simulink model "AEB_Gateway_Only"  (Simulink 9.2)
settings: Solver=FixedStepDiscrete  StartTime=0.0  StopTime=inf  FixedStep=0.05  RelTol=1e-3
PostLoadFcn:
  | , if any(exist('dsrtsu_mdlpostloadfcn', 'file') == [2, 3, 6]), try dsrtsu_mdlpostloadfcn('Execute', bdroot); catch fprintf('Error in PostLoadFcn (dsrtsu_mdlpostloadfcn) for model "%s":\n %s\n', bdroot, lasterr); end, end,
libraries: rtican x7
(part 1 of 2)
settings Model: DSRTSU_INTERNAL_RTI_VER=520  DSRTSU_INTERNAL_RTI_TYPE=rti1401  RTICANMMDATA=struct('GeneralSetupData',struct('modelroot','C:\Users\cordunoalbarran\Documents\dSPACE\ControlDesk\6.3\AEB_Pac_testing\AEB_shortlist','generalsettings',struct('filesettings',struct('destfolder',struct('Name','RTICANMM_FILES','Check',1),'buildfolder',struct('Name','.','Check',1),'AbsDestfolder',struct('Name','C:\Users\cordunoalbarran\Documents\dSPACE\ControlDesk\6.3\AEB_Pac_testing\AEB_shortlist\RTICANMM_FILES'),'AbsBuildfolder',struct('Name','C:\Users\cordunoalbarran\Documents\dSPACE\ControlDesk\6.3\AEB_Pac_testing\AEB_shortlist'))),'options',struct('addpaths',1,'rmpaths',1,'addtrcexclusion',logical(1),'cannavigator',struct('checkmonitoring',0),'show_usrtrc',0,'use_usrtrc',0),'advanced',struct('options',ones(1,100)),'MPSetup',{{}},'RTI',struct('Type','RTI1401','Ver','7.10','Date','02-May-2018'),'modelname','AEB_Gateway_Only','block','AEB_Gateway_Only'))  DSRTSU_INTERNAL_RTIFPGA=110  Creator=ffearon  LastModifiedBy=cordunoalbarran
settings DataIOCC: LimitDataPoints=off  SaveFormat=Dataset  SignalLoggingSaveFormat=Dataset
settings OptimizationCC: BlockReduction=off  LifeSpan=auto
settings DebuggingCC: UnderspecifiedInitializationDetection=Simplified  MergeDetectMultiDrivingBlocksExec=error  FcnCallInpInsideContextMsg=error  StateNameClashWarn=none  SFUnexpectedBacktrackingDiag=error  SFNoUnconditionalDefaultTransitionDiag=error  SFExecutionAtInitializationDiag=warning
settings HardwareCC: ProdLargestAtomicInteger=Integer  ProdLargestAtomicFloat=Float  ProdIntDivRoundTo=Zero  ProdEndianess=BigEndian  ProdHWDeviceType=Custom Processor->Custom  TargetIntDivRoundTo=Zero  TargetEndianess=BigEndian  TargetHWDeviceType=Custom Processor->Custom
settings ModelReferenceCC: PropagateSignalLabelsOutOfModel=on
settings SFSimCC: SimUseLocalCustomCode=on  MATLABDynamicMemAlloc=off
settings RTWCC: SystemTargetFile=rti1401.tlc  MakeCommand=make_rti  TemplateMakefile=rti1401.tmf  Description=dSPACE DS1401 Hardware Platform  RTWUseLocalCustomCode=on
settings CodeAppCC: StateflowObjectComments=off
settings STFCustomTargetCC: ParMdlRefBuildCompliant=on  GRTInterface=off  SystemTargetFile=rti1401.tlc
settings GRTTargetCC: CompOptLevelCompliant=off  ConcurrentExecutionCompliant=off  GeneratePreprocessorConditionals=Use local settings  MatFileLogging=off  CPPClassGenCompliant=off  GRTInterface=off  UseToolchainInfoCompliant=off
settings CustomProperty: DataType=RTWOptions_EnumType_C__Program Files_dSPACE RCPHIL 2018-A_MATLAB_RTI_RTI1401_TLC_rti1401_1InitialSimState  Value=RUN
settings EnumStrPairs: String=RUN
settings ConfigComp: CovMetricSettings=dwe  CovHtmlReporting=off  CovSaveCumulativeToWorkspaceVar=off  CovSaveSingleToWorkspaceVar=off  CovExternalEMLEnable=on

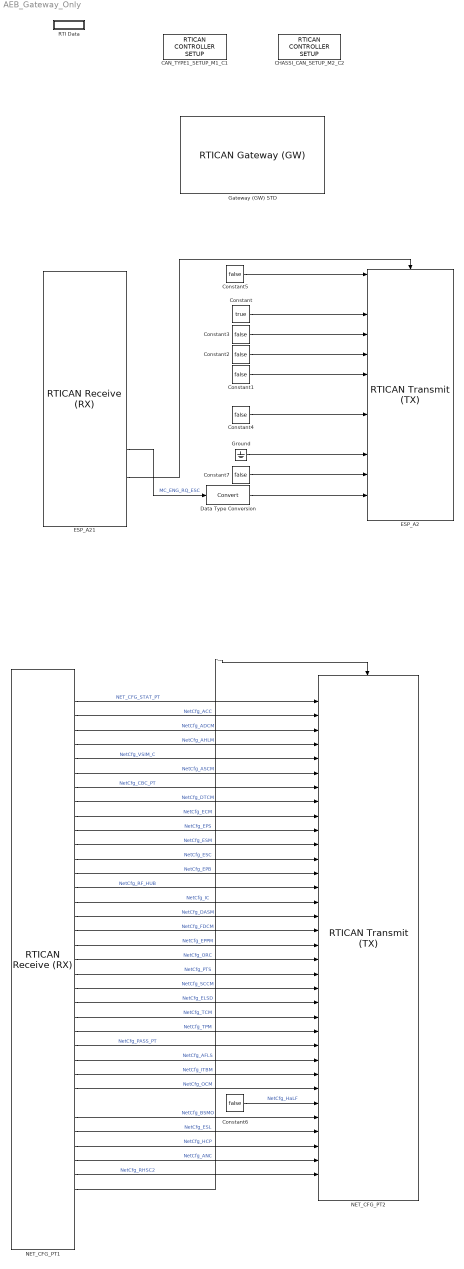
== system AEB_Gateway_Only ==
  CAN_TYPE1_SETUP_M1_C1 : rtican/RTICAN CONTROLLER SETUP   Reserved1=[]  Reserved2=[]  Reserved3=[]  Reserved4=[]  AcceptanceMask=[]  ArbitrationField=[]  Parameters=[]  SFcnRTICANSettings=[]  MS_Struct=[]  BoardTypeNo=[]  BoardNo=[]  ChannelNo=[]  DialogFcn=[]  UnitName=[]  Revision=[]  UnitValues=[]  DSProperties=struct('RTI',struct('Version',uint32(12),'BlockType',struct('isSLSource',uint8(0),'isSLSink',uint8(0),'isHWSource',uint8(0),'isHWSink',uint8(0),'isSetup',uint8(1),'isInline',uint8(1),'isNonInline',uint8(0),'isInterrupt',uint8(0),'isChannelwise',uint8(0)),'IOBoardType','RTICAN','UnitType','NON_MESSAGE','Identifier','MASTER','DialogType','ML','BlockSet','RTICAN','SlaveProcessor','CAN'))  RTIBlockInterface=struct('InputPortsWidth',int32(0),'InputPortsActive',0,'OutputPortsWidth',int32(0),'OutputPortsActive',0,'DialogFcn','rtican_master_setup_gui','BlockDisplay',{{['CAN CONTROLLER\n SETUP'],'center'}},'IconTransparency','on','InitLevel',3,'IWork',{{{'',uint32(2)}}},'BlockName',struct('Token',{{'CAN_TYPE','_SETUP_M','_C'}},'BlockParam',{{'BoardTypeNo','BoardNo','ChannelNo'}}),'ParameterTunableNames',{{}})  RTIBlockParameters="struct('BoardTypeNo',{{1,'OFF',[]}},'BoardNo',{{1,'ON',[1 16]}},'ChannelNo',{{1,'ON',[1 2]}},'AcceptanceMask',{{0,'OFF',[]}},'ArbitrationField',{{0,'OFF',[]}},'Parameters',{{struct('Config',struct('Baudrate',500,'SampleMode',1,'UsedParamSet',1,'validSettings',1,'isBTRvalues',0,'Advanced',struct('Baudrate',{500,500,500},'Frequency',{24000000,36000000,64000000},'Settings',{struct('SMPL',0,'BRP',0,'NBT',24,'TSEG1',15,'TSEG2',6,'SJW',3,'SP',70),struct('SMPL',0,'BRP',1,'NBT',18,'TSEG1',14,'TSEG2',1,'SJW',1,'SP',88),struct('SMPL',0,'BRP',3,'NBT',16,'TSEG1',12,'TSEG2',1,'SJW',1,'SP',87)},'BTR0',{192,65,67},'BTR1',{111,30,28})),'configType',1,'Options',struct('DataFileSelected',1,'DataFileName',{{['..\\..\\..\\..\\..\\..\\..\\..\\intrepidcs\\pacifica dbc\\e4a_r4_ccan_cr11690_mod.dbc']}},'DataFileDate',{{['26-Feb-2019 09:25:05']}},'InterfaceFcn','rtican_dbc_file_parser','InterfaceFcnFileName','','LabelConfigType','volatile','AcceptanceMaskSelected',0,'MsgDataType','SgnSpecification','NumType','hex','MaskType','STD','AcceptanceMask',0,'ArbitrationField',0,'UseMultipleMessageAccess',1),'RxReceiveStdOptions',struct('RxServiceStdEnabled',1,'RxServiceStdMsgIdent',1000,'RxServiceStdIdentNumType',1,'RxServiceStdIdentMask',0,'RxServiceStdMaskNumType',1,'RxServiceStdQueueSize',256),'RxReceiveXtdOptions',struct('RxServiceXtdEnabled',0,'RxServiceXtdMsgIdent',1001,'RxServiceXtdIdentNumType',1,'RxServiceXtdIdentMask',0,'RxServiceXtdMaskNumType',1,'RxServiceXtdQueueSize',64),'PartialNetworkingOptions',struct('switchedon',0,'format',1,'idmask',['    XXXXX XXXXXXXX XXXXXXXX XXXXXXXX'],'idcode','0','idfilter','0','datamaskused',0,'datalength',1,'datamask','0x0000000000000000','partialnetworkenable',0),'general',struct('Termination_common',1,'Termination_C252',1,'BusConfigurationRegister',0,'Transceiver','ISO11898','isFromLib',0)),'OFF',[]}},'CCPParameters',{{struct('CRO',struct('Format','STD','NumFormat','hex','Id',1639),'DTO',struct('Format','STD','NumFormat','hex','Id',2017),'StationAdr',struct('NumFormat','hex','Value',57),'StationId',struct('Value',['dSPACE CCP Service']),'Enabled',0),'OFF',[]}},'XCPParameters',{{struct('MASTER',struct('Format','STD','NumFormat','hex','Id',256),'SLAVE',struct('Format','STD','NumFormat','hex','Id',510),'Enabled',0,'PIDTransmissionEnabled',0),'OFF',[]}},'GroupId',{{struct('Group',{{'RTICAN'}},'No',1,'Behavior',{{'EVER'}},'BlockType',{{'SOURCE'}},'NameChangeFlag',1),'OFF',[]}},'SFcnRTICANSettings',{{struct('Baudrate',500,'configType',1,'AdvancedConfig',struct('Frequency',{},'BTR0',{},'BTR1',{}),'UsedParamSet',1,'STDMaskSelected','no','XTDMaskSelected','no','BoardType','DS1','BoardNo',1,'ControllerNo',1,'Transceiver','ISO11898','BusConfigRegister',0,'TerminationRes',120,'UseMultipleMessageAccess','yes','STDRXSrvcUsed','yes','STDRXSrvcMsgId',1,'STDRXSrvcMsgMask',0,'STDRXSrvcQueueSize',256,'XTDRXSrvcUsed','no','XTDRXSrvcMsgId',1001,'XTDRXSrvcQueueSize',64,'XTDRXSrvcMsgMask',0,'PN_IsPNTransciever',0,'PN_IsPNEnabled',0,'PN_MsgFormat',1,'PN_idcode',0,'PN_idmask',2047,'PN_datamaskused',0,'PN_datalength',0,'PN_datamask',['0xFF, 0xFF, 0xFF, 0xFF, 0xFF, 0xFF, 0xFF, 0xFF']),'OFF',[]}},'SFcnRTICCPSettings',{{struct('CRO',struct('Format','STD','NumFormat','hex','Id',1639),'DTO',struct('Format','STD','NumFormat','hex','Id',2017),'StationAdr',struct('NumFormat','hex','Value',57),'StationId',struct('Value',['dSPACE CCP Service']),'Enabled',0),'OFF',[]}},'SFcnRTIXCPSettings',{{struct('MASTER',struct('Format','STD','NumFormat','hex','Id',256),'SLAVE',struct('Format','STD','NumFormat','hex','Id',510),'Enabled',0,'PIDTransmissionEnabled',0),'OFF',[]}},'TLCFileName',{{'rtican_master_setup','OFF',[]}})"  RTISFcnParameters=struct('SFcnRTICANSettings','struct','SFcnRTICCPSettings','struct','SFcnRTIXCPSettings','struct','AcceptanceMask','int32','ArbitrationField','int32','TLCFileName','char')  RTIBlockParaDefault="struct('BoardTypeNo',4302,'BoardNo',1,'ChannelNo',1,'AcceptanceMask',0,'ArbitrationField',0,'Parameters',struct('Config',struct('Baudrate',500,'SampleMode',1,'UsedParamSet',1,'validSettings',1,'isBTRvalues',0,'Advanced',struct('Frequency',16000000,'BTR0',64,'BTR1',28,'Settings',struct('SMPL',0,'BRP',0,'NBT',16,'TSEG1',12,'TSEG2',1,'SJW',1,'SP',87))),'configType',1,'Options',struct('DataFileSelected',0,'DataFileName',{{['<no datafile support>']}},'DataFileDate',{{''}},'InterfaceFcn','rtican_dbc_file_parser','InterfaceFcnFileName','','LabelConfigType','volatile','AcceptanceMaskSelected',0,'MsgDataType','AllwaysDouble','NumType','hex','MaskType','STD','AcceptanceMask',0,'ArbitrationField',0,'UseMultipleMessageAccess',0),'RxReceiveStdOptions',struct('RxServiceStdEnabled',0,'RxServiceStdMsgIdent',1000,'RxServiceStdIdentNumType',1,'RxServiceStdIdentMask',0,'RxServiceStdMaskNumType',1,'RxServiceStdQueueSize',64),'RxReceiveXtdOptions',struct('RxServiceXtdEnabled',0,'RxServiceXtdMsgIdent',1001,'RxServiceXtdIdentNumType',1,'RxServiceXtdIdentMask',0,'RxServiceXtdMaskNumType',1,'RxServiceXtdQueueSize',64),'PartialNetworkingOptions',struct('switchedon',0,'format',1,'idmask',['    XXXXX XXXXXXXX XXXXXXXX XXXXXXXX'],'idcode','0','idfilter','0','datamaskused',0,'datalength',1,'datamask','0x0000000000000000','partialnetworkenable',0),'general',struct('Termination_common',1,'Termination_C252',1,'BusConfigurationRegister',0,'Transceiver','ISO11898','isFromLib',1)),'CCPParameters',struct('CRO',struct('Format','STD','NumFormat','hex','Id',1639),'DTO',struct('Format','STD','NumFormat','hex','Id',2017),'StationAdr',struct('NumFormat','hex','Value',57),'StationId',struct('Value',['dSPACE CCP Service']),'Enabled',0),'XCPParameters',struct('MASTER',struct('Format','STD','NumFormat','hex','Id',256),'SLAVE',struct('Format','STD','NumFormat','hex','Id',510),'Enabled',0,'PIDTransmissionEnabled',0),'GroupId',struct('Group',{{'RTICAN'}},'No',1,'Behavior',{{'EVER'}},'BlockType',{{'SOURCE'}},'NameChangeFlag',1),'SFcnRTICANSettings',struct('Baudrate',500,'configType',1,'AdvandedConfig',struct('Frequency',16000000,'BTR0','0x40','BTR1','0x1C'),'UsedParamSet',1,'STDMaskSelected','no','XTDMaskSelected','no','BoardType','DS4302','BoardNo',1,'ControllerNo',1,'Transceiver','ISO11898','BusConfigRegister',0,'TerminationRes',120,'UseMultipleMessageAccess','no','STDRXSrvcUsed','no','STDRXSrvcMsgId',1000,'STDRXSrvcMsgMask',0,'STDRXSrvcQueueSize',64,'XTDRXSrvcUsed','no','XTDRXSrvcMsgId',1001,'XTDRXSrvcQueueSize',64,'XTDRXSrvcMsgMask',0),'SFcnRTICCPSettings',struct('CRO',struct('Format','STD','NumFormat','hex','Id',1639),'DTO',struct('Format','STD','NumFormat','hex','Id',2017),'StationAdr',struct('NumFormat','hex','Value',57),'StationId',struct('Value',['dSPACE CCP Service']),'Enabled',0),'SFcnRTIXCPSettings',struct('MASTER',struct('Format','STD','NumFormat','hex','Id',256),'SLAVE',struct('Format','STD','NumFormat','hex','Id',510),'Enabled',0,'PIDTransmissionEnabled',0),'TLCFileName','rtican_master_setup')"
      settings: AttributesFormatString=Group Id: RTICAN1\n  SourceProductName=dSPACE RTI CAN Blockset
  CHASSI_CAN_SETUP_M2_C2 : rtican/RTICAN CONTROLLER SETUP   Reserved1=[]  Reserved2=[]  Reserved3=[]  Reserved4=[]  AcceptanceMask=[]  ArbitrationField=[]  Parameters=[]  SFcnRTICANSettings=[]  MS_Struct=[]  BoardTypeNo=[]  BoardNo=[]  ChannelNo=[]  DialogFcn=[]  UnitName=[]  Revision=[]  UnitValues=[]  DSProperties=struct('RTI',struct('Version',uint32(12),'BlockType',struct('isSLSource',uint8(0),'isSLSink',uint8(0),'isHWSource',uint8(0),'isHWSink',uint8(0),'isSetup',uint8(1),'isInline',uint8(1),'isNonInline',uint8(0),'isInterrupt',uint8(0),'isChannelwise',uint8(0)),'IOBoardType','RTICAN','UnitType','NON_MESSAGE','Identifier','MASTER','DialogType','ML','BlockSet','RTICAN','SlaveProcessor','CAN'))  RTIBlockInterface=struct('InputPortsWidth',int32(0),'InputPortsActive',0,'OutputPortsWidth',int32(0),'OutputPortsActive',0,'DialogFcn','rtican_master_setup_gui','BlockDisplay',{{['CAN CONTROLLER\n SETUP'],'center'}},'IconTransparency','on','InitLevel',3,'IWork',{{{'',uint32(2)}}},'BlockName',struct('Token',{{'CAN_TYPE','_SETUP_M','_C'}},'BlockParam',{{'BoardTypeNo','BoardNo','ChannelNo'}}),'ParameterTunableNames',{{}})  RTIBlockParameters="struct('BoardTypeNo',{{1,'OFF',[]}},'BoardNo',{{2,'ON',[1 16]}},'ChannelNo',{{2,'ON',[1 2]}},'AcceptanceMask',{{0,'OFF',[]}},'ArbitrationField',{{0,'OFF',[]}},'Parameters',{{struct('Config',struct('Baudrate',500,'SampleMode',1,'UsedParamSet',1,'validSettings',1,'isBTRvalues',0,'Advanced',struct('Baudrate',{500,500,500},'Frequency',{24000000,36000000,64000000},'Settings',{struct('SMPL',0,'BRP',0,'NBT',24,'TSEG1',15,'TSEG2',6,'SJW',3,'SP',70),struct('SMPL',0,'BRP',1,'NBT',18,'TSEG1',14,'TSEG2',1,'SJW',1,'SP',88),struct('SMPL',0,'BRP',3,'NBT',16,'TSEG1',12,'TSEG2',1,'SJW',1,'SP',87)},'BTR0',{192,65,67},'BTR1',{111,30,28})),'configType',1,'Options',struct('DataFileSelected',1,'DataFileName',{{['..\\..\\..\\..\\..\\..\\..\\..\\intrepidcs\\pacifica dbc\\e4a_r4_ccan_cr11690_mod.dbc']}},'DataFileDate',{{['26-Feb-2019 09:25:05']}},'InterfaceFcn','rtican_dbc_file_parser','InterfaceFcnFileName','','LabelConfigType','volatile','AcceptanceMaskSelected',0,'MsgDataType','SgnSpecification','NumType','hex','MaskType','STD','AcceptanceMask',0,'ArbitrationField',0,'UseMultipleMessageAccess',1),'RxReceiveStdOptions',struct('RxServiceStdEnabled',1,'RxServiceStdMsgIdent',1000,'RxServiceStdIdentNumType',1,'RxServiceStdIdentMask',0,'RxServiceStdMaskNumType',1,'RxServiceStdQueueSize',256),'RxReceiveXtdOptions',struct('RxServiceXtdEnabled',0,'RxServiceXtdMsgIdent',1001,'RxServiceXtdIdentNumType',1,'RxServiceXtdIdentMask',0,'RxServiceXtdMaskNumType',1,'RxServiceXtdQueueSize',64),'PartialNetworkingOptions',struct('switchedon',0,'format',1,'idmask',['    XXXXX XXXXXXXX XXXXXXXX XXXXXXXX'],'idcode','0','idfilter','0','datamaskused',0,'datalength',1,'datamask','0x0000000000000000','partialnetworkenable',0),'general',struct('Termination_common',1,'Termination_C252',1,'BusConfigurationRegister',0,'Transceiver','ISO11898','isFromLib',0)),'OFF',[]}},'CCPParameters',{{struct('CRO',struct('Format','STD','NumFormat','hex','Id',1639),'DTO',struct('Format','STD','NumFormat','hex','Id',2017),'StationAdr',struct('NumFormat','hex','Value',57),'StationId',struct('Value',['dSPACE CCP Service']),'Enabled',0),'OFF',[]}},'XCPParameters',{{struct('MASTER',struct('Format','STD','NumFormat','hex','Id',256),'SLAVE',struct('Format','STD','NumFormat','hex','Id',510),'Enabled',0,'PIDTransmissionEnabled',0),'OFF',[]}},'GroupId',{{struct('Group',{{'RTICAN'}},'No',3,'Behavior',{{'EVER'}},'BlockType',{{'SOURCE'}},'NameChangeFlag',1),'OFF',[]}},'SFcnRTICANSettings',{{struct('Baudrate',500,'configType',1,'AdvancedConfig',struct('Frequency',{},'BTR0',{},'BTR1',{}),'UsedParamSet',1,'STDMaskSelected','no','XTDMaskSelected','no','BoardType','DS1','BoardNo',2,'ControllerNo',2,'Transceiver','ISO11898','BusConfigRegister',0,'TerminationRes',120,'UseMultipleMessageAccess','yes','STDRXSrvcUsed','yes','STDRXSrvcMsgId',1,'STDRXSrvcMsgMask',0,'STDRXSrvcQueueSize',256,'XTDRXSrvcUsed','no','XTDRXSrvcMsgId',1001,'XTDRXSrvcQueueSize',64,'XTDRXSrvcMsgMask',0,'PN_IsPNTransciever',0,'PN_IsPNEnabled',0,'PN_MsgFormat',1,'PN_idcode',0,'PN_idmask',2047,'PN_datamaskused',0,'PN_datalength',0,'PN_datamask',['0xFF, 0xFF, 0xFF, 0xFF, 0xFF, 0xFF, 0xFF, 0xFF']),'OFF',[]}},'SFcnRTICCPSettings',{{struct('CRO',struct('Format','STD','NumFormat','hex','Id',1639),'DTO',struct('Format','STD','NumFormat','hex','Id',2017),'StationAdr',struct('NumFormat','hex','Value',57),'StationId',struct('Value',['dSPACE CCP Service']),'Enabled',0),'OFF',[]}},'SFcnRTIXCPSettings',{{struct('MASTER',struct('Format','STD','NumFormat','hex','Id',256),'SLAVE',struct('Format','STD','NumFormat','hex','Id',510),'Enabled',0,'PIDTransmissionEnabled',0),'OFF',[]}},'TLCFileName',{{'rtican_master_setup','OFF',[]}})"  RTISFcnParameters=struct('SFcnRTICANSettings','struct','SFcnRTICCPSettings','struct','SFcnRTIXCPSettings','struct','AcceptanceMask','int32','ArbitrationField','int32','TLCFileName','char')  RTIBlockParaDefault="struct('BoardTypeNo',4302,'BoardNo',1,'ChannelNo',1,'AcceptanceMask',0,'ArbitrationField',0,'Parameters',struct('Config',struct('Baudrate',500,'SampleMode',1,'UsedParamSet',1,'validSettings',1,'isBTRvalues',0,'Advanced',struct('Frequency',16000000,'BTR0',64,'BTR1',28,'Settings',struct('SMPL',0,'BRP',0,'NBT',16,'TSEG1',12,'TSEG2',1,'SJW',1,'SP',87))),'configType',1,'Options',struct('DataFileSelected',0,'DataFileName',{{['<no datafile support>']}},'DataFileDate',{{''}},'InterfaceFcn','rtican_dbc_file_parser','InterfaceFcnFileName','','LabelConfigType','volatile','AcceptanceMaskSelected',0,'MsgDataType','AllwaysDouble','NumType','hex','MaskType','STD','AcceptanceMask',0,'ArbitrationField',0,'UseMultipleMessageAccess',0),'RxReceiveStdOptions',struct('RxServiceStdEnabled',0,'RxServiceStdMsgIdent',1000,'RxServiceStdIdentNumType',1,'RxServiceStdIdentMask',0,'RxServiceStdMaskNumType',1,'RxServiceStdQueueSize',64),'RxReceiveXtdOptions',struct('RxServiceXtdEnabled',0,'RxServiceXtdMsgIdent',1001,'RxServiceXtdIdentNumType',1,'RxServiceXtdIdentMask',0,'RxServiceXtdMaskNumType',1,'RxServiceXtdQueueSize',64),'PartialNetworkingOptions',struct('switchedon',0,'format',1,'idmask',['    XXXXX XXXXXXXX XXXXXXXX XXXXXXXX'],'idcode','0','idfilter','0','datamaskused',0,'datalength',1,'datamask','0x0000000000000000','partialnetworkenable',0),'general',struct('Termination_common',1,'Termination_C252',1,'BusConfigurationRegister',0,'Transceiver','ISO11898','isFromLib',1)),'CCPParameters',struct('CRO',struct('Format','STD','NumFormat','hex','Id',1639),'DTO',struct('Format','STD','NumFormat','hex','Id',2017),'StationAdr',struct('NumFormat','hex','Value',57),'StationId',struct('Value',['dSPACE CCP Service']),'Enabled',0),'XCPParameters',struct('MASTER',struct('Format','STD','NumFormat','hex','Id',256),'SLAVE',struct('Format','STD','NumFormat','hex','Id',510),'Enabled',0,'PIDTransmissionEnabled',0),'GroupId',struct('Group',{{'RTICAN'}},'No',1,'Behavior',{{'EVER'}},'BlockType',{{'SOURCE'}},'NameChangeFlag',1),'SFcnRTICANSettings',struct('Baudrate',500,'configType',1,'AdvandedConfig',struct('Frequency',16000000,'BTR0','0x40','BTR1','0x1C'),'UsedParamSet',1,'STDMaskSelected','no','XTDMaskSelected','no','BoardType','DS4302','BoardNo',1,'ControllerNo',1,'Transceiver','ISO11898','BusConfigRegister',0,'TerminationRes',120,'UseMultipleMessageAccess','no','STDRXSrvcUsed','no','STDRXSrvcMsgId',1000,'STDRXSrvcMsgMask',0,'STDRXSrvcQueueSize',64,'XTDRXSrvcUsed','no','XTDRXSrvcMsgId',1001,'XTDRXSrvcQueueSize',64,'XTDRXSrvcMsgMask',0),'SFcnRTICCPSettings',struct('CRO',struct('Format','STD','NumFormat','hex','Id',1639),'DTO',struct('Format','STD','NumFormat','hex','Id',2017),'StationAdr',struct('NumFormat','hex','Value',57),'StationId',struct('Value',['dSPACE CCP Service']),'Enabled',0),'SFcnRTIXCPSettings',struct('MASTER',struct('Format','STD','NumFormat','hex','Id',256),'SLAVE',struct('Format','STD','NumFormat','hex','Id',510),'Enabled',0,'PIDTransmissionEnabled',0),'TLCFileName','rtican_master_setup')"
      settings: AttributesFormatString=Group Id: RTICAN3\n  SourceProductName=dSPACE RTI CAN Blockset
  Constant : Constant  Value=true
  Constant{1..7} (7 alike) : Constant  Value=false
  Data Type Conversion : DataTypeConversion
  ESP_A2 : rtican/RTICAN Transmit (TX)   Reserved1=[]  Reserved2=[]  Reserved3=[]  Reserved4=[]  SfcnMessage=[]  Msg_Struct=[]  BoardTypeNo=[]  BoardNo=[]  ChannelNo=[]  Parameters=[]  DialogFcn=[]  UnitName=[]  Revision=[]  UnitValues=[]  DSProperties=struct('RTI',struct('Version',uint32(5),'BlockType',struct('isSLSource',uint8(1),'isSLSink',uint8(1),'isHWSource',uint8(0),'isHWSink',uint8(0),'isSetup',uint8(0),'isInline',uint8(1),'isNonInline',uint8(0),'isInterrupt',uint8(0),'isChannelwise',uint8(0)),'IOBoardType','RTICAN','UnitType','MESSAGE','Identifier','TX','DialogType','MSVC','BlockSet','RTICAN','SlaveProcessor','CAN'))  RTIBlockInterface=struct('InputPortsWidth',int32([1 1 1 1 1 1 1 1 1 1 1 1 1]),'InputPortsActive',ones(1,13),'InputPortsName',{{'EngTrq_Rq_ESC','MaxTrqGrdAvail_ESC','DAS_Enbl_Rq','ASRActive','EngTrqMin_Rq_ESC','EngTrqMax_Rq_ESC','MaxTqAvail_ESC','PrefillActive','VehicleSpeed_SSM','DAS_RqActv','Brk_Jrk_Rsp','MC_ENG_RQ_ESC','CRC_ENG_RQ_ESC'}},'InputPortsDataType',{{'SS_BOOLEAN','SS_UINT16','SS_BOOLEAN','SS_BOOLEAN','SS_BOOLEAN','SS_BOOLEAN','SS_INT32','SS_BOOLEAN','SS_DOUBLE','SS_UINT8','SS_BOOLEAN','SS_UINT8','SS_UINT8'}},'OutputPortsWidth',int32([1 1 1 1]),'OutputPortsActive',[1 1 1 1],'OutputPortsName',{{['TX status'],['TX time'],['TX delta time'],['TX delay time']}},'DialogFcn','rtican_message_interface_gui','BlockDisplay',{{'','center'}},'IconTransparency','on','InitLevel',3,'BlockName',struct('Token',{{'ESP_A2'}}),'SampleTime',{{-1}},'TriggerPort',{{'none'}},'EnablePort',{{'yes'}})  RTIBlockParameters=struct('BoardTypeNo',{{1,'OFF',[]}},'BoardNo',{{2,'ON',[1 16]}},'ChannelNo',{{2,'ON',[1 2]}},'Parameters',{{struct('DataFileSupport',struct('DataFileSelectedMaster',1,'DataFileSelectedLocal',1,'DataFileName',['c:\users\cordunoalbarran\documents\repo\avcampari\guv0 dbcs\lyftctrlcan.dbc|'],'DataFileDate',['26-Feb-2019 09:25:05'],'SelectedFile',['..\..\..\..\..\..\..\..\intrepidcs\pacifica dbc\e4a_r4_ccan_cr11690_mod.dbc'],'InterfaceFcn','rtican_dbc_file_parser'),'Options',struct('StatusSelected',1,'TimeSelected',1,'DeltaTimeSelected',1,'DelayTimeSelected',1,'DelayTimeTXCommandSelected',0,'EncodeSetUnusedBitsToOne',0,'EnableMsgLoopback',0,'TriggerPort',struct('Selected',0,'TriggerType',0),'EnablePortSelected',1,'SignalOnPortnameSelected',1,'UserCoding',struct('Selected',1,'InterfaceFile','UserEncodingFile','FcnName','Message_CRC_Encoder','InportSelected',0,'InportWidth',1,'OutportSelected',0,'OutportWidth',1),'TerminationMsg',struct('Selected',0,'Byte0_7','0'),'InitialMsg',struct('Selected',0,'Byte0_7','0')),'Message',struct('MsgOnBlocknameSelected',1,'MsgName','ESP_A2','MsgIdFormat',0,'MsgId',268,'MsgLength',8,'NumSignals',13,'SampleTime',-1,'StartTime',struct('Selected',0,'Value',9),'AutoRepeatTime',struct('Selected',0,'Value',0.1),'Timeout',struct('Selected',0,'Value',0.1),'DelayTime',struct('Selected',0,'Value',0.1),'Signal',struct('SgnName',{'EngTrq_Rq_ESC','MaxTrqGrdAvail_ESC','DAS_Enbl_Rq','ASRActive','EngTrqMin_Rq_ESC','EngTrqMax_Rq_ESC','MaxTqAvail_ESC','PrefillActive','VehicleSpeed_SSM','DAS_RqActv','Brk_Jrk_Rsp','MC_ENG_RQ_ESC','CRC_ENG_RQ_ESC'},'SgnStartBit',{6,16,20,21,22,23,32,34,48,48,51,52,56},'SgnLength',{1,10,1,1,1,1,10,1,14,3,1,4,8},'ByteLayout',{0,2,0,0,0,0,2,0,2,0,0,0,0},'Factor',{1,64,1,1,1,1,64,1,2^-6,1,1,1,1},'Offset',{0,0,0,0,0,0,-65472,0,0,0,0,0,0},'SgnComment',{['DUMMY Signal Not Used on EVA'],'',['DUMMY Signal Not Used on EVA'],['Traction control is active'],['DUMMY Signal Not Used on EVA'],['DUMMY Signal Not Used on EVA'],'',['Brake prefill is active - True = [1]'],'',['DAS request active'],['Brake jerk response; True = [1]'],['Message counter'],['CRC-checksum byte 1 to 7 according to SAE J1850']},'SgnUnit',{'','Nm/s','','','','','Nm','','km/h','','','',''},'Min',{0,0,0,0,0,0,-65472,0,0,0,0,0,0},'Max',{0,65472,0,0,0,0,0,0,255.98,0,0,15,0},'SgnType',{0,0,0,0,0,0,0,0,0,0,0,0,0},'SLDataType',{'SS_BOOLEAN','SS_UINT16','SS_BOOLEAN','SS_BOOLEAN','SS_BOOLEAN','SS_BOOLEAN','SS_INT32','SS_BOOLEAN','SS_DOUBLE','SS_UINT8','SS_BOOLEAN','SS_UINT8','SS_UINT8'},'DataType',{0,0,0,0,0,0,0,0,0,0,0,0,0},'ModeValue',{-1,-1,-1,-1,-1,-1,-1,-1,-1,-1,-1,-1,-1}),'MsgIdNumFormat',0,'MsgComment',{{''}}),'Version',1.2,'general',struct('isFromLib',0)),'OFF',[]}},'GroupId',{{struct('Group',{{'RTICAN'}},'No',3,'Behavior',{{'NAMECHANGE'}},'BlockType',{{'SINK'}},'NameChangeFlag',0),'OFF',[]}},'SFcnRTICANMessage',{{struct('MsgType','TX','SFcnPortType','Scalar','MsgName','ESP_A2','MsgIdFormat','STD','MsgId',268,'MsgLength',8,'NumSignals',13,'SampleTime',-1,'StartTime',struct('Selected','no','Value',9),'AutoRepeatTime',struct('Selected','no','Value',0.1),'Timeout',struct('Selected','no','Value',0.1),'Signal',struct('SgnName',{'EngTrq_Rq_ESC','MaxTrqGrdAvail_ESC','DAS_Enbl_Rq','ASRActive','EngTrqMin_Rq_ESC','EngTrqMax_Rq_ESC','MaxTqAvail_ESC','PrefillActive','VehicleSpeed_SSM','DAS_RqActv','Brk_Jrk_Rsp','MC_ENG_RQ_ESC','CRC_ENG_RQ_ESC'},'SgnStartBit',{6,16,20,21,22,23,32,34,48,48,51,52,56},'SgnLength',{1,10,1,1,1,1,10,1,14,3,1,4,8},'ByteLayout',{['little endian'],['motorola back.'],['little endian'],['little endian'],['little endian'],['little endian'],['motorola back.'],['little endian'],['motorola back.'],['little endian'],['little endian'],['little endian'],['little endian']},'Factor',{1,64,1,1,1,1,64,1,2^-6,1,1,1,1},'Offset',{0,0,0,0,0,0,-65472,0,0,0,0,0,0},'SgnType',{'standard','standard','standard','standard','standard','standard','standard','standard','standard','standard','standard','standard','standard'},'SLDataType',{'SS_BOOLEAN','SS_UINT16','SS_BOOLEAN','SS_BOOLEAN','SS_BOOLEAN','SS_BOOLEAN','SS_INT32','SS_BOOLEAN','SS_DOUBLE','SS_UINT8','SS_BOOLEAN','SS_UINT8','SS_UINT8'},'DataType',{['unsigned int'],['unsigned int'],['unsigned int'],['unsigned int'],['unsigned int'],['unsigned int'],['unsigned int'],['unsigned int'],['unsigned int'],['unsigned int'],['unsigned int'],['unsigned int'],['unsigned int']},'ModeValue',{-1,-1,-1,-1,-1,-1,-1,-1,-1,-1,-1,-1,-1}),'StatusSelected','yes','TimeSelected','yes','DeltaTimeSelected','yes','DelayTimeSelected','yes','DelayTimeTXCommandSelected','no','EncodeSetUnusedBitsToOne','no','EnableMsgLoopback','no','TriggerPort',struct('Selected','no','TriggerType',0),'EnablePortSelected','yes','UserCoding',struct('Selected','yes','InterfaceFile','UserEncodingFile','FcnName','Message_CRC_Encoder','InportSelected','no','InportWidth',1,'OutportSelected','no','OutportWidth',1),'TerminationMsg',struct('Selected','no','Byte0','0x00','Byte1','0x00','Byte2','0x00','Byte3','0x00','Byte4','0x00','Byte5','0x00','Byte6','0x00','Byte7','0x00'),'InitialMsg',struct('Selected','no','Byte0','0x00','Byte1','0x00','Byte2','0x00','Byte3','0x00','Byte4','0x00','Byte5','0x00','Byte6','0x00','Byte7','0x00'),'BoardType','DS1','BoardNo',2,'ControllerNo',2),'OFF',[]}},'TLCFileName',{{'rtican_tx_message','OFF',[]}})  RTISFcnParameters=struct('SFcnRTICANMessage','struct','TLCFileName','char')  RTIBlockParaDefault=struct('BoardTypeNo',4302,'BoardNo',1,'ChannelNo',1,'Parameters',struct('DataFileSupport',struct('DataFileSelectedMaster',0,'DataFileSelectedLocal',0,'DataFileName','','DataFileDate','','SelectedFile',['<no file selected>']),'Options',struct('StatusSelected',1,'TimeSelected',1,'DeltaTimeSelected',1,'DelayTimeSelected',1,'DelayTimeTXCommandSelected',0,'EncodeSetUnusedBitsToOne',0,'EnableMsgLoopback',0,'TriggerPort',struct('Selected',0,'TriggerType','rising'),'EnablePortSelected',0,'SignalOnPortnameSelected',1,'UserCoding',struct('Selected',0,'InterfaceFile','UserEncodingFile','FcnName','UserEncodeFcn','InportSelected',0,'InportWidth',1,'OutportSelected',0,'OutportWidth',1),'TerminationMsg',struct('Selected',0,'Byte0_7','0'),'InitialMsg',struct('Selected',0,'Byte0_7','0')),'Message',struct('MsgOnBlocknameSelected',0,'MsgName',['TX Message'],'MsgIdFormat',0,'MsgId',100,'MsgLength',8,'NumSignals',1,'SampleTime',-1,'StartTime',struct('Selected',0,'Value',0),'AutoRepeatTime',struct('Selected',0,'Value',0.1),'Timeout',struct('Selected',0,'Value',0.1),'DelayTime',struct('Selected',0,'Value',0.1),'Signal',struct('SgnName',['TX signal'],'SgnStartBit',0,'SgnLength',8,'SgnType',0,'ModeValue',-1,'DataType',0,'SLDataType','SS_DOUBLE','ByteLayout',0,'Factor',1,'Offset',0,'Min',0,'Max',255,'SgnComment',{{}},'SgnUnit',''),'MsgIdNumFormat',0,'MsgComment',{{''}}),'Version',1.2,'general',struct('isFromLib',1)),'GroupId',struct('Group',{{'RTICAN'}},'No',1,'Behavior',{{'NAMECHANGE'}},'BlockType',{{'SINK'}},'NameChangeFlag',0),'SFcnRTICANMessage',struct('MsgType','TX','MsgName',['TX Message'],'MsgIdFormat','STD','MsgId',100,'MsgLength',2,'NumSignals',1,'SampleTime',-1,'StartTime',struct('Selected','no','Value',0),'AutoRepeatTime',struct('Selected','no','Value',0.1),'Timeout',struct('Selected','no','Value',0.1),'DelayTime',struct('Selected','no','Value',0.1),'Signal',struct('SgnName',['TX signal'],'SgnStartBit',0,'SgnLength',8,'SgnType','standard','ModeValue',-1,'DataType',['unsigned int'],'ByteLayout',['little endian'],'SLDataType','SS_DOUBLE','Factor',1,'Offset',0),'StatusSelected','yes','TimeSelected','yes','DeltaTimeSelected','yes','DelayTimeSelected','yes','EnablePortSelected','no','EnableMsgLoopback','no','DelayTimeTXCommandSelected','no','EncodeSetUnusedBitsToOne','no','UserCoding',struct('Selected','no','InterfaceFile','UserDecodingFile','FcnName','UserDecodeFcn','InportSelected','no','InportWidth',1,'OutportSelected','no','OutportWidth',1),'TerminationMsg',struct('Selected','no','Byte0','0x00','Byte1','0x00','Byte2','0x00','Byte3','0x00','Byte4','0x00','Byte5','0x00','Byte6','0x00','Byte7','0x00'),'InitialMsg',struct('Selected','no','Byte0','0x00','Byte1','0x00','Byte2','0x00','Byte3','0x00','Byte4','0x00','Byte5','0x00','Byte6','0x00','Byte7','0x00'),'TriggerPort',struct('Selected','no','TriggerType','rising'),'BoardType','DS4302','BoardNo',1,'ControllerNo',1,'SFcnPortType','Scalar'),'TLCFileName','rtican_tx_message')
      settings: AttributesFormatString=Group Id: RTICAN3\n  SourceProductName=dSPACE RTI CAN Blockset
  ESP_A21 : rtican/RTICAN Receive (RX)   Reserved1=[]  Reserved2=[]  Reserved3=[]  Reserved4=[]  SfcnMessage=[]  Msg_Struct=[]  BoardTypeNo=[]  BoardNo=[]  ChannelNo=[]  Parameters=[]  DialogFcn=[]  UnitName=[]  Revision=[]  UnitValues=[]  DSProperties=struct('RTI',struct('Version',uint32(5),'BlockType',struct('isSLSource',uint8(1),'isSLSink',uint8(1),'isHWSource',uint8(0),'isHWSink',uint8(0),'isSetup',uint8(0),'isInline',uint8(1),'isNonInline',uint8(0),'isInterrupt',uint8(0),'isChannelwise',uint8(0)),'IOBoardType','RTICAN','UnitType','MESSAGE','Identifier','RX','DialogType','MSVC','BlockSet','RTICAN','SlaveProcessor','CAN'))  RTIBlockInterface=struct('OutputPortsWidth',int32([1 1 1 1 1 1 1 1 1 1 1 1 1 1 1 1]),'OutputPortsActive',ones(1,16),'OutputPortsName',{{'EngTrq_Rq_ESC','MaxTrqGrdAvail_ESC','DAS_Enbl_Rq','ASRActive','EngTrqMin_Rq_ESC','EngTrqMax_Rq_ESC','MaxTqAvail_ESC','PrefillActive','VehicleSpeed_SSM','DAS_RqActv','Brk_Jrk_Rsp','MC_ENG_RQ_ESC','CRC_ENG_RQ_ESC',['RX status'],['RX time'],['RX delta time']}},'OutputPortsDataType',{{'SS_BOOLEAN','SS_UINT16','SS_BOOLEAN','SS_BOOLEAN','SS_BOOLEAN','SS_BOOLEAN','SS_INT32','SS_BOOLEAN','SS_DOUBLE','SS_UINT8','SS_BOOLEAN','SS_UINT8','SS_UINT8','SS_DOUBLE','SS_DOUBLE','SS_DOUBLE'}},'OutputPortsLabel',{{'EngTrq_Rq_ESC','MaxTrqGrdAvail_ESC','DAS_Enbl_Rq','ASRActive','EngTrqMin_Rq_ESC','EngTrqMax_Rq_ESC','MaxTqAvail_ESC','PrefillActive','VehicleSpeed_SSM','DAS_RqActv','Brk_Jrk_Rsp','MC_ENG_RQ_ESC','CRC_ENG_RQ_ESC','','',''}},'OutputPortsLabelMode','ON','InputPortsWidth',int32(0),'InputPortsActive',0,'DialogFcn','rtican_message_interface_gui','BlockDisplay',{{'','center'}},'IconTransparency','on','ParameterTunableNames',{{}},'InitLevel',3,'BlockName',struct('Token',{{'ESP_A2'}}),'SampleTime',{{-1}},'TriggerPort',{{'none'}},'EnablePort',{{'none'}})  RTIBlockParameters=struct('BoardTypeNo',{{1,'OFF',[]}},'BoardNo',{{1,'ON',[1 16]}},'ChannelNo',{{1,'ON',[1 2]}},'Parameters',{{struct('DataFileSupport',struct('DataFileSelectedMaster',1,'DataFileSelectedLocal',1,'DataFileName',['c:\intrepidcs\pacifica dbc\e4a_r4_ccan_cr11690_mod.dbc|'],'DataFileDate',['26-Feb-2019 09:25:05'],'SelectedFile',['..\..\..\..\..\..\..\..\intrepidcs\pacifica dbc\e4a_r4_ccan_cr11690_mod.dbc'],'InterfaceFcn','rtican_dbc_file_parser'),'Options',struct('StatusSelected',1,'TimeSelected',1,'DeltaTimeSelected',1,'BytePortSelected',0,'MessageLengthSelected',0,'TriggerPort',struct('Selected',0,'TriggerType',0),'UserCoding',struct('Selected',0,'InterfaceFile','UserDecodingFile','FcnName','UserDecodeFcn','InportSelected',0,'InportWidth',1,'OutportSelected',0,'OutportWidth',1),'EnablePortSelected',0,'SignalOnPortnameSelected',1,'UseRXService',0),'Message',struct('MsgOnBlocknameSelected',1,'MsgName','ESP_A2','MsgIdFormat',0,'MsgId',268,'MsgLength',8,'NumSignals',13,'SampleTime',-1,'Signal',struct('SgnName',{'EngTrq_Rq_ESC','MaxTrqGrdAvail_ESC','DAS_Enbl_Rq','ASRActive','EngTrqMin_Rq_ESC','EngTrqMax_Rq_ESC','MaxTqAvail_ESC','PrefillActive','VehicleSpeed_SSM','DAS_RqActv','Brk_Jrk_Rsp','MC_ENG_RQ_ESC','CRC_ENG_RQ_ESC'},'SgnStartBit',{6,16,20,21,22,23,32,34,48,48,51,52,56},'SgnLength',{1,10,1,1,1,1,10,1,14,3,1,4,8},'SgnType',{0,0,0,0,0,0,0,0,0,0,0,0,0},'ModeValue',{-1,-1,-1,-1,-1,-1,-1,-1,-1,-1,-1,-1,-1},'DataType',{0,0,0,0,0,0,0,0,0,0,0,0,0},'ByteLayout',{0,2,0,0,0,0,2,0,2,0,0,0,0},'Factor',{1,64,1,1,1,1,64,1,2^-6,1,1,1,1},'Offset',{0,0,0,0,0,0,-65472,0,0,0,0,0,0},'SgnComment',{{['DUMMY Signal Not Used on EVA']},{''},{['DUMMY Signal Not Used on EVA']},{['Traction control is active']},{['DUMMY Signal Not Used on EVA']},{['DUMMY Signal Not Used on EVA']},{''},{['Brake prefill is active - True = [1]']},{''},{['DAS request active']},{['Brake jerk response; True = [1]']},{['Message counter']},{['CRC-checksum byte 1 to 7 according to SAE J1850']}},'SgnUnit',{'','Nm/s','','','','','Nm','','km/h','','','',''},'Min',{0,0,0,0,0,0,-65472,0,0,0,0,0,0},'Max',{0,65472,0,0,0,0,0,0,255.98,0,0,15,0},'SLDataType',{'SS_BOOLEAN','SS_UINT16','SS_BOOLEAN','SS_BOOLEAN','SS_BOOLEAN','SS_BOOLEAN','SS_INT32','SS_BOOLEAN','SS_DOUBLE','SS_UINT8','SS_BOOLEAN','SS_UINT8','SS_UINT8'}),'MsgIdNumFormat',0,'MsgComment',{{''}}),'Version',1.2,'general',struct('isFromLib',0)),'OFF',[]}},'GroupId',{{struct('Group',{{'RTICAN'}},'No',1,'Behavior',{{'NAMECHANGE'}},'BlockType',{{'SINK'}},'NameChangeFlag',0),'OFF',[]}},'SFcnRTICANMessage',{{struct('MsgType','RX','SFcnPortType','Scalar','MsgName','ESP_A2','MsgIdFormat','STD','MsgId',268,'MsgLength',8,'NumSignals',13,'SampleTime',-1,'Signal',struct('SgnName',{'EngTrq_Rq_ESC','MaxTrqGrdAvail_ESC','DAS_Enbl_Rq','ASRActive','EngTrqMin_Rq_ESC','EngTrqMax_Rq_ESC','MaxTqAvail_ESC','PrefillActive','VehicleSpeed_SSM','DAS_RqActv','Brk_Jrk_Rsp','MC_ENG_RQ_ESC','CRC_ENG_RQ_ESC'},'SgnStartBit',{6,16,20,21,22,23,32,34,48,48,51,52,56},'SgnLength',{1,10,1,1,1,1,10,1,14,3,1,4,8},'SgnType',{'standard','standard','standard','standard','standard','standard','standard','standard','standard','standard','standard','standard','standard'},'ModeValue',{-1,-1,-1,-1,-1,-1,-1,-1,-1,-1,-1,-1,-1},'DataType',{['unsigned int'],['unsigned int'],['unsigned int'],['unsigned int'],['unsigned int'],['unsigned int'],['unsigned int'],['unsigned int'],['unsigned int'],['unsigned int'],['unsigned int'],['unsigned int'],['unsigned int']},'ByteLayout',{['little endian'],['motorola back.'],['little endian'],['little endian'],['little endian'],['little endian'],['motorola back.'],['little endian'],['motorola back.'],['little endian'],['little endian'],['little endian'],['little endian']},'Factor',{1,64,1,1,1,1,64,1,2^-6,1,1,1,1},'Offset',{0,0,0,0,0,0,-65472,0,0,0,0,0,0},'SLDataType',{'SS_BOOLEAN','SS_UINT16','SS_BOOLEAN','SS_BOOLEAN','SS_BOOLEAN','SS_BOOLEAN','SS_INT32','SS_BOOLEAN','SS_DOUBLE','SS_UINT8','SS_BOOLEAN','SS_UINT8','SS_UINT8'}),'StatusSelected','yes','TimeSelected','yes','DeltaTimeSelected','yes','BytePortSelected','no','MessageLengthSelected','no','TriggerPort',struct('Selected','no','TriggerType',0),'UserCoding',struct('Selected','no','InterfaceFile','UserDecodingFile','FcnName','UserDecodeFcn','InportSelected','no','InportWidth',1,'OutportSelected','no','OutportWidth',1),'EnablePortSelected','no','UseRXService','no','BoardType','DS1','BoardNo',1,'ControllerNo',1),'OFF',[]}},'TLCFileName',{{'rtican_rx_message','OFF',[]}})  RTISFcnParameters=struct('SFcnRTICANMessage','struct','TLCFileName','char')  RTIBlockParaDefault=struct('BoardTypeNo',4302,'BoardNo',1,'ChannelNo',1,'Parameters',struct('DataFileSupport',struct('DataFileSelectedMaster',0,'DataFileSelectedLocal',0,'DataFileName','','DataFileDate','','SelectedFile',['<no file selected>']),'Options',struct('StatusSelected',1,'TimeSelected',1,'DeltaTimeSelected',1,'BytePortSelected',0,'MessageLengthSelected',0,'TriggerPort',struct('Selected',0,'TriggerType','rising'),'UserCoding',struct('Selected',0,'InterfaceFile','UserDecodingFile','FcnName','UserDecodeFcn','InportSelected',0,'InportWidth',1,'OutportSelected',0,'OutportWidth',1),'EnablePortSelected',0,'SignalOnPortnameSelected',1,'UseRXService',0),'Message',struct('MsgOnBlocknameSelected',0,'MsgName',['RX Message'],'MsgIdFormat',0,'MsgId',100,'MsgLength',8,'NumSignals',1,'SampleTime',-1,'Signal',struct('SgnName',['RX signal'],'SgnStartBit',0,'SgnLength',8,'SgnType',0,'ModeValue',-1,'DataType',0,'SLDataType','SS_DOUBLE','ByteLayout',0,'Factor',1,'Offset',0,'Min',0,'Max',255,'SgnComment',{{}},'SgnUnit',''),'MsgIdNumFormat',0,'MsgComment',{{''}}),'Version',1.2,'general',struct('isFromLib',1)),'GroupId',struct('Group',{{'RTICAN'}},'No',1,'Behavior',{{'NAMECHANGE'}},'BlockType',{{'SINK'}},'NameChangeFlag',0),'SFcnRTICANMessage',struct('MsgType','RX','MsgName',['RX Message'],'MsgIdFormat','STD','MsgId',100,'MsgLength',8,'NumSignals',1,'SampleTime',-1,'Signal',struct('SgnName',['RX signal'],'SgnStartBit',0,'SgnLength',8,'SgnType','standard','ModeValue',-1,'DataType',['unsigned int'],'ByteLayout',['little endian'],'SLDataType','SS_DOUBLE','Factor',1,'Offset',0),'StatusSelected','yes','TimeSelected','yes','DeltaTimeSelected','yes','BytePortSelected','no','MessageLengthSelected','no','EnablePortSelected','no','UserCoding',struct('Selected','no','InterfaceFile','UserDecodingFile','FcnName','UserDecodeFcn','InportSelected','no','InportWidth',1,'OutportSelected','no','OutportWidth',1),'TriggerPort',struct('Selected','no','TriggerType','rising'),'UseRXService','no','BoardType','DS4302','BoardNo',1,'ControllerNo',1,'SFcnPortType','Scalar'),'TLCFileName','rtican_rx_message')
      settings: AttributesFormatString=Group Id: RTICAN1\n  SourceProductName=dSPACE RTI CAN Blockset
  Gateway (GW) STD : rtican/RTICAN Gateway (GW)  Reserved1=[]  Reserved2=[]  Reserved3=[]  Reserved4=[]  BoardTypeNo=[]  BoardNo=[]  ChannelNo=[]  BoardTypeNo2=[]  BoardNo2=[]  ChannelNo2=[]  Parameters=[]  DialogFcn=[]  UnitName=[]  Revision=[]  UnitValues=[]  DSProperties=struct('RTI',struct('Version',uint32(1),'BlockType',struct('isSLSource',uint8(1),'isSLSink',uint8(1),'isHWSource',uint8(0),'isHWSink',uint8(0),'isSetup',uint8(0),'isInline',uint8(1),'isNonInline',uint8(0),'isInterrupt',uint8(0),'isChannelwise',uint8(0)),'IOBoardType','RTICAN','UnitType','MESSAGE','Identifier','GW','DialogType','MSVC','BlockSet','RTICAN','SlaveProcessor','CAN'))  RTIBlockInterface=struct('OutputPortsWidth',int32([1 1 1 1]),'OutputPortsActive',[1 1 1 1],'OutputPortsName',{{['RX count 1'],['TX count 1'],['RX count 2'],['TX count 2']}},'OutputPortsDataType',{{'SS_DOUBLE','SS_DOUBLE','SS_DOUBLE','SS_DOUBLE'}},'OutputPortsLabel',{{'','','',''}},'OutputPortsLabelMode','off','InitLevel',3,'DialogFcn','rtican_gateway_interface_gui','BlockDisplay',{{['DS1 B1 C1\n <==>\nDS1 B2 C2'],'center'}},'IconTransparency','on','IWork',{{{'',uint32(4)}}},'BlockName',struct('Token',{{['Gateway (GW) STD']}}),'SampleTime',{{-1}},'TriggerPort',{{'none'}},'EnablePort',{{'none'}})  RTIBlockParameters=struct('BoardTypeNo',{{1,'OFF',[]}},'BoardNo',{{1,'ON',[1 16]}},'ChannelNo',{{1,'ON',[1 2]}},'BoardTypeNo2',{{1,'OFF',[]}},'BoardNo2',{{2,'ON',[1 16]}},'ChannelNo2',{{2,'ON',[1 4]}},'MessageIDFormat',{{'STD','OFF',[]}},'Parameters',{{struct('SampleTime',-1,'DataFileSupport',struct('DataFileSelectedMaster',1,'DataFileSelectedLocal',0,'DataFileName',['c:\intrepidcs\pacifica dbc\e4a_r4_ccan_cr11690_mod.dbc|'],'DataFileDate','','SelectedFile',['..\..\..\..\..\..\..\..\intrepidcs\pacifica dbc\e4a_r4_ccan_cr11690_mod.dbc']),'Options',struct('RXCnt1Selected',1,'TXCnt1Selected',1,'RXCnt2Selected',1,'TXCnt2Selected',1,'BothDirSelected',1,'DiffListsSelected',1,'MsgIdFormat',0,'TriggerPort',struct('Selected',0,'TriggerType',0),'EnablePortSelected',0),'ExcludeList12',struct('Count',257,'MsgList',struct('MsgId',{969,1788,1729,1787,1784,1754,1736,1737,1786,1730,1758,1732,1762,1728,1763,838,523,524,525,998,999,927,937,520,564,861,624,456,856,848,500,499,501,625,2015,860,1900,1898,2023,2020,1568,1899,2019,2016,1882,1864,1865,2018,1858,1902,1886,1860,1890,1856,1891,1150,1260,1258,2031,2028,1284,1235,1259,2027,2024,1242,1224,1225,2026,1252,1218,1262,1246,1220,1250,1216,1251,1151,653,864,850,880,896,912,928,936,632,779,703,863,308,290,672,257,1468,1409,1427,1467,1464,1434,1416,1417,1466,1444,1410,1438,1412,1442,1408,1443,522,463,268,736,737,682,1016,989,988,987,986,985,707,714,715,1017,1018,1019,1020,1021,1022,1023,991,1008,983,982,981,980,979,706,709,710,1009,1010,1011,1012,1014,1015,984,908,974,901,639,853,854,799,798,817,579,705,678,658,729,704,654,878,560,832,782,938,939,940,941,942,943,958,959,517,515,516,518,956,926,1025,1083,1050,1031,1032,1082,1026,1024,1033,1059,464,466,469,294,542,764,766,859,532,584,900,826,608,825,671,388,448,924,656,521,929,746,857,858,1596,1537,1555,1595,1592,1562,1544,1545,1594,1572,1538,1566,1540,1570,1536,1571,879,719,557,808,773,526,527,376,698,1100,906,1004,1005,1006,1007,1099,1101,898,907,947,949,948,950,2047},'MsgName',{'AMB_TEMP_DISP','APPL_ECU_BSMO','APPL_ECU_CBC','APPL_ECU_EBCM','APPL_ECU_ECM','APPL_ECU_EPS','APPL_ECU_ESL','APPL_ECU_ESM','APPL_ECU_HCP','APPL_ECU_IC','APPL_ECU_OCM','APPL_ECU_ORC','APPL_ECU_PTS','APPL_ECU_RF_HUB','APPL_ECU_SCCM','AS_CHIME_STAT','BCM_CODE_ESL_REQUEST','BCM_CODE_TRM_REQUEST','BCM_MINICRYPT_ACK','BU_NET_CFG_INT','BU_NET_CFG_PT','BU_NET_CFG_ePT','CBC_CFG1','CBC_PT6','CBC_PT7','CBC_PT7_IBS2','CBC_PT8','CBC_VTA','COMPASS_A1','Clock_Date','DAS_A3','DAS_A3_A','DAS_A4','DAS_A5','DG_RQ_GLOBAL','DIRECT_INFO','D_RQ_AHCP','D_RQ_APM','D_RQ_BPCM','D_RQ_BSMO','D_RQ_CBC','D_RQ_EAC','D_RQ_EBCM','D_RQ_ECM','D_RQ_EPS','D_RQ_ESL','D_RQ_ESM','D_RQ_HCP','D_RQ_IC','D_RQ_OBCM','D_RQ_OCM','D_RQ_ORC','D_RQ_PTS','D_RQ_RF_HUB','D_RQ_SCCM','D_RQ_SGW','D_RS_AHCP','D_RS_APM','D_RS_BPCM','D_RS_BSMO','D_RS_CBC','D_RS_DASM','D_RS_EAC','D_RS_EBCM','D_RS_ECM','D_RS_EPS','D_RS_ESL','D_RS_ESM','D_RS_HCP','D_RS_HaLF','D_RS_IC','D_RS_OBCM','D_RS_OCM','D_RS_ORC','D_RS_PTS','D_RS_RF_HUB','D_RS_SCCM','D_RS_SGW','EBCM_C1','ECM_APPL1','ECM_APPL2','ECM_APPL3','ECM_APPL4','ECM_APPL5','ECM_APPL6','ECM_APPL7','ECM_B2','ECM_B5','ECM_B7','ECM_B8','ECM_CRUISE_MAP','ECM_GEAR','ECM_INDICATORS','ECM_SKIM_OBD','ECU_APPL_BSMO','ECU_APPL_CBC','ECU_APPL_DASM','ECU_APPL_EBCM','ECU_APPL_ECM','ECU_APPL_EPS','ECU_APPL_ESL','ECU_APPL_ESM','ECU_APPL_HCP','ECU_APPL_HaLF','ECU_APPL_IC','ECU_APPL_OCM','ECU_APPL_ORC','ECU_APPL_PTS','ECU_APPL_RF_HUB','ECU_APPL_SCCM','EPS_SDS_Resp','ESL_CODE_RESPONSE','ESP_A2','ESP_B1','ESP_B2','ESP_B5','EcuBuCfg1','EcuBuCfg10','EcuBuCfg11','EcuBuCfg12','EcuBuCfg13','EcuBuCfg14','EcuBuCfg15','EcuBuCfg16','EcuBuCfg17','EcuBuCfg2','EcuBuCfg3','EcuBuCfg4','EcuBuCfg5','EcuBuCfg6','EcuBuCfg7','EcuBuCfg8','EcuBuCfg9','EcuCfg1','EcuCfg10','EcuCfg11','EcuCfg12','EcuCfg13','EcuCfg14','EcuCfg15','EcuCfg16','EcuCfg17','EcuCfg2','EcuCfg3','EcuCfg4','EcuCfg5','EcuCfg7','EcuCfg8','EcuCfg9','GPS_POS3','GW_Dev','GW_IBS2_DATA','GW_IBS_DATA','GW_LIN_I_C1','GW_LIN_I_C1_IBS2','GW_LIN_I_C2','GW_LIN_I_C2_IBS2','GW_LIN_I_C3','GW_LIN_I_C4','GW_LIN_I_C5','HALF_HMI_STATUS','HALF_MTO_SteerControl','HALF_SWVM_CTRL','HCP_2','HCP_C1','HCP_DISP','HVAC_A2','IC_500Cyc','IC_A5','IC_TripData_1','IC_TripData_2','IC_TripData_3','IC_TripData_4','IC_TripData_5','IC_TripData_6','IC_TripData_7','IC_TripData_8','IMMO_CODE_REQUEST','IMMO_CODE_REQUEST_HCP','IMMO_CODE_RESPONSE','IMMO_CODE_RESPONSE_HCP','NAV_DATA','NET_CFG_EPT','NM_CBC','NM_EBCM','NM_EPS','NM_ESC','NM_ESL','NM_HCP','NM_IC','NM_RF_HUB','NM_SBWM','NM_SCCM','ORC_A1','ORC_A2','ORC_A4','ORC_YRS_DATA','ORC_YRS_INFO','PCM_EDR','PCM_EDR2','PN14_IBS2_DATA','PN14_IBS_DATA','PN14_STAT','PN14_STAT_IBS2','PTS_1','PTS_2','PTS_CHIME_STAT','PTS_StrCtrl','RFHUB_A1','RFHUB_A2','RFHUB_A3','RF_CHAR','RHSC_SDS_SteerControl','Radio_A3','SBW_ROT1','SDS_CBC_CMD','SDS_CBC_STAT','SD_RS_BSMO','SD_RS_CBC','SD_RS_DASM','SD_RS_EBCM','SD_RS_ECM','SD_RS_EPS','SD_RS_ESL','SD_RS_ESM','SD_RS_HCP','SD_RS_HaLF','SD_RS_IC','SD_RS_OCM','SD_RS_ORC','SD_RS_PTS','SD_RS_RF_HUB','SD_RS_SCCM','STATUS_C_ESL','STATUS_C_PTS','SWS_8','TGW_DATA_IC','TPM_A2','TRM_CODE_RESPONSE','TRM_MKP_KEY','TRNS_STAT2','Uconnect_1','VehCfg6','VehCfg8','VehCfgBu1','VehCfgBu2','VehCfgBu3','VehCfgBu4','VehCfgBu5','VehCfgBu6','VehCfgBu7','VehCfgBu8','VehCfgCSM1','VehCfgCSM1_BU','VehCfgCSM2','VehCfgCSM2_BU','WAKE_SGW'},'FromDBC',{1,1,1,1,1,1,1,1,1,1,1,1,1,1,1,1,1,1,1,1,1,1,1,1,1,1,1,1,1,1,1,1,1,1,1,1,1,1,1,1,1,1,1,1,1,1,1,1,1,1,1,1,1,1,1,1,1,1,1,1,1,1,1,1,1,1,1,1,1,1,1,1,1,1,1,1,1,1,1,1,1,1,1,1,1,1,1,1,1,1,1,1,1,1,1,1,1,1,1,1,1,1,1,1,1,1,1,1,1,1,1,1,1,1,1,1,1,1,1,1,1,1,1,1,1,1,1,1,1,1,1,1,1,1,1,1,1,1,1,1,1,1,1,1,1,1,1,1,1,1,1,1,1,1,1,1,1,1,1,1,1,1,1,1,1,1,1,1,1,1,1,1,1,1,1,1,1,1,1,1,1,1,1,1,1,1,1,1,1,1,1,1,1,1,1,1,1,1,1,1,1,1,1,1,1,1,1,1,1,1,1,1,1,1,1,1,1,1,1,1,1,1,1,1,1,1,1,1,1,1,1,1,1,1,1,1,1,1,1,1,1,1,1,1,1,1,1,1,1,1,1,1,1,1,1,1,1})),'ExcludeList21',struct('Count',0,'MsgList',struct('MsgId',0,'MsgName','empty','FromDBC',0)),'Version',1,'general',struct('isFromLib',0,'BoardType2',1,'BoardNo2',2,'ControllerNo2',2,'GroupId2',struct('Group','RTICAN','No',3))),'OFF',[]}},'GroupId',{{struct('Group',{{'RTICAN'}},'No',1,'Behavior',{{'NAMECHANGE'}},'BlockType',{{'SINK'}},'NameChangeFlag',0),'OFF',[]}},'GroupId2',{{struct('Group',{{'RTICAN'}},'No',3,'Behavior',{{'NAMECHANGE'}},'BlockType',{{'SINK'}},'NameChangeFlag',0),'OFF',[]}},'SFcnRTICANMessage',{{struct('MsgIdFormat','STD','SampleTime',-1,'RXCnt1Selected','yes','TXCnt1Selected','yes','RXCnt2Selected','yes','TXCnt2Selected','yes','BothDirSelected','yes','DiffListsSelected','yes','EnablePortSelected','no','TriggerPort',struct('Selected','no','TriggerType','rising'),'ExcludeList12',struct('Count',257,'MsgList',struct('MsgId',{969,1788,1729,1787,1784,1754,1736,1737,1786,1730,1758,1732,1762,1728,1763,838,523,524,525,998,999,927,937,520,564,861,624,456,856,848,500,499,501,625,2015,860,1900,1898,2023,2020,1568,1899,2019,2016,1882,1864,1865,2018,1858,1902,1886,1860,1890,1856,1891,1150,1260,1258,2031,2028,1284,1235,1259,2027,2024,1242,1224,1225,2026,1252,1218,1262,1246,1220,1250,1216,1251,1151,653,864,850,880,896,912,928,936,632,779,703,863,308,290,672,257,1468,1409,1427,1467,1464,1434,1416,1417,1466,1444,1410,1438,1412,1442,1408,1443,522,463,268,736,737,682,1016,989,988,987,986,985,707,714,715,1017,1018,1019,1020,1021,1022,1023,991,1008,983,982,981,980,979,706,709,710,1009,1010,1011,1012,1014,1015,984,908,974,901,639,853,854,799,798,817,579,705,678,658,729,704,654,878,560,832,782,938,939,940,941,942,943,958,959,517,515,516,518,956,926,1025,1083,1050,1031,1032,1082,1026,1024,1033,1059,464,466,469,294,542,764,766,859,532,584,900,826,608,825,671,388,448,924,656,521,929,746,857,858,1596,1537,1555,1595,1592,1562,1544,1545,1594,1572,1538,1566,1540,1570,1536,1571,879,719,557,808,773,526,527,376,698,1100,906,1004,1005,1006,1007,1099,1101,898,907,947,949,948,950,2047},'MsgName',{'AMB_TEMP_DISP','APPL_ECU_BSMO','APPL_ECU_CBC','APPL_ECU_EBCM','APPL_ECU_ECM','APPL_ECU_EPS','APPL_ECU_ESL','APPL_ECU_ESM','APPL_ECU_HCP','APPL_ECU_IC','APPL_ECU_OCM','APPL_ECU_ORC','APPL_ECU_PTS','APPL_ECU_RF_HUB','APPL_ECU_SCCM','AS_CHIME_STAT','BCM_CODE_ESL_REQUEST','BCM_CODE_TRM_REQUEST','BCM_MINICRYPT_ACK','BU_NET_CFG_INT','BU_NET_CFG_PT','BU_NET_CFG_ePT','CBC_CFG1','CBC_PT6','CBC_PT7','CBC_PT7_IBS2','CBC_PT8','CBC_VTA','COMPASS_A1','Clock_Date','DAS_A3','DAS_A3_A','DAS_A4','DAS_A5','DG_RQ_GLOBAL','DIRECT_INFO','D_RQ_AHCP','D_RQ_APM','D_RQ_BPCM','D_RQ_BSMO','D_RQ_CBC','D_RQ_EAC','D_RQ_EBCM','D_RQ_ECM','D_RQ_EPS','D_RQ_ESL','D_RQ_ESM','D_RQ_HCP','D_RQ_IC','D_RQ_OBCM','D_RQ_OCM','D_RQ_ORC','D_RQ_PTS','D_RQ_RF_HUB','D_RQ_SCCM','D_RQ_SGW','D_RS_AHCP','D_RS_APM','D_RS_BPCM','D_RS_BSMO','D_RS_CBC','D_RS_DASM','D_RS_EAC','D_RS_EBCM','D_RS_ECM','D_RS_EPS','D_RS_ESL','D_RS_ESM','D_RS_HCP','D_RS_HaLF','D_RS_IC','D_RS_OBCM','D_RS_OCM','D_RS_ORC','D_RS_PTS','D_RS_RF_HUB','D_RS_SCCM','D_RS_SGW','EBCM_C1','ECM_APPL1','ECM_APPL2','ECM_APPL3','ECM_APPL4','ECM_APPL5','ECM_APPL6','ECM_APPL7','ECM_B2','ECM_B5','ECM_B7','ECM_B8','ECM_CRUISE_MAP','ECM_GEAR','ECM_INDICATORS','ECM_SKIM_OBD','ECU_APPL_BSMO','ECU_APPL_CBC','ECU_APPL_DASM','ECU_APPL_EBCM','ECU_APPL_ECM','ECU_APPL_EPS','ECU_APPL_ESL','ECU_APPL_ESM','ECU_APPL_HCP','ECU_APPL_HaLF','ECU_APPL_IC','ECU_APPL_OCM','ECU_APPL_ORC','ECU_APPL_PTS','ECU_APPL_RF_HUB','ECU_APPL_SCCM','EPS_SDS_Resp','ESL_CODE_RESPONSE','ESP_A2','ESP_B1','ESP_B2','ESP_B5','EcuBuCfg1','EcuBuCfg10','EcuBuCfg11','EcuBuCfg12','EcuBuCfg13','EcuBuCfg14','EcuBuCfg15','EcuBuCfg16','EcuBuCfg17','EcuBuCfg2','EcuBuCfg3','EcuBuCfg4','EcuBuCfg5','EcuBuCfg6','EcuBuCfg7','EcuBuCfg8','EcuBuCfg9','EcuCfg1','EcuCfg10','EcuCfg11','EcuCfg12','EcuCfg13','EcuCfg14','EcuCfg15','EcuCfg16','EcuCfg17','EcuCfg2','EcuCfg3','EcuCfg4','EcuCfg5','EcuCfg7','EcuCfg8','EcuCfg9','GPS_POS3','GW_Dev','GW_IBS2_DATA','GW_IBS_DATA','GW_LIN_I_C1','GW_LIN_I_C1_IBS2','GW_LIN_I_C2','GW_LIN_I_C2_IBS2','GW_LIN_I_C3','GW_LIN_I_C4','GW_LIN_I_C5','HALF_HMI_STATUS','HALF_MTO_SteerControl','HALF_SWVM_CTRL','HCP_2','HCP_C1','HCP_DISP','HVAC_A2','IC_500Cyc','IC_A5','IC_TripData_1','IC_TripData_2','IC_TripData_3','IC_TripData_4','IC_TripData_5','IC_TripData_6','IC_TripData_7','IC_TripData_8','IMMO_CODE_REQUEST','IMMO_CODE_REQUEST_HCP','IMMO_CODE_RESPONSE','IMMO_CODE_RESPONSE_HCP','NAV_DATA','NET_CFG_EPT','NM_CBC','NM_EBCM','NM_EPS','NM_ESC','NM_ESL','NM_HCP','NM_IC','NM_RF_HUB','NM_SBWM','NM_SCCM','ORC_A1','ORC_A2','ORC_A4','ORC_YRS_DATA','ORC_YRS_INFO','PCM_EDR','PCM_EDR2','PN14_IBS2_DATA','PN14_IBS_DATA','PN14_STAT','PN14_STAT_IBS2','PTS_1','PTS_2','PTS_CHIME_STAT','PTS_StrCtrl','RFHUB_A1','RFHUB_A2','RFHUB_A3','RF_CHAR','RHSC_SDS_SteerControl','Radio_A3','SBW_ROT1','SDS_CBC_CMD','SDS_CBC_STAT','SD_RS_BSMO','SD_RS_CBC','SD_RS_DASM','SD_RS_EBCM','SD_RS_ECM','SD_RS_EPS','SD_RS_ESL','SD_RS_ESM','SD_RS_HCP','SD_RS_HaLF','SD_RS_IC','SD_RS_OCM','SD_RS_ORC','SD_RS_PTS','SD_RS_RF_HUB','SD_RS_SCCM','STATUS_C_ESL','STATUS_C_PTS','SWS_8','TGW_DATA_IC','TPM_A2','TRM_CODE_RESPONSE','TRM_MKP_KEY','TRNS_STAT2','Uconnect_1','VehCfg6','VehCfg8','VehCfgBu1','VehCfgBu2','VehCfgBu3','VehCfgBu4','VehCfgBu5','VehCfgBu6','VehCfgBu7','VehCfgBu8','VehCfgCSM1','VehCfgCSM1_BU','VehCfgCSM2','VehCfgCSM2_BU','WAKE_SGW'},'FromDBC',{1,1,1,1,1,1,1,1,1,1,1,1,1,1,1,1,1,1,1,1,1,1,1,1,1,1,1,1,1,1,1,1,1,1,1,1,1,1,1,1,1,1,1,1,1,1,1,1,1,1,1,1,1,1,1,1,1,1,1,1,1,1,1,1,1,1,1,1,1,1,1,1,1,1,1,1,1,1,1,1,1,1,1,1,1,1,1,1,1,1,1,1,1,1,1,1,1,1,1,1,1,1,1,1,1,1,1,1,1,1,1,1,1,1,1,1,1,1,1,1,1,1,1,1,1,1,1,1,1,1,1,1,1,1,1,1,1,1,1,1,1,1,1,1,1,1,1,1,1,1,1,1,1,1,1,1,1,1,1,1,1,1,1,1,1,1,1,1,1,1,1,1,1,1,1,1,1,1,1,1,1,1,1,1,1,1,1,1,1,1,1,1,1,1,1,1,1,1,1,1,1,1,1,1,1,1,1,1,1,1,1,1,1,1,1,1,1,1,1,1,1,1,1,1,1,1,1,1,1,1,1,1,1,1,1,1,1,1,1,1,1,1,1,1,1,1,1,1,1,1,1,1,1,1,1,1,1})),'ExcludeList21',struct('Count',0,'MsgList',struct('MsgId',0,'MsgName','empty','FromDBC',0)),'BoardTypeNo',int32([1 1]),'BoardNo',int32([1 2]),'ControllerNo',int32([1 2]),'SFcnPortType','Scalar'),'OFF',[]}},'TLCFileName',{{'rtican_gw_message','OFF',[]}})  RTISFcnParameters=struct('SFcnRTICANMessage','struct','TLCFileName','char')  RTIBlockParaDefault=struct('BoardTypeNo',4302,'BoardNo',1,'ChannelNo',1,'BoardTypeNo2',4302,'BoardNo2',1,'ChannelNo2',2,'MessageIDFormat','STD','Parameters',struct('SampleTime',-1,'DataFileSupport',struct('DataFileSelectedMaster',0,'DataFileSelectedLocal',0,'DataFileName','','DataFileDate','','SelectedFile',['<no file selected>']),'Options',struct('RXCnt1Selected',0,'TXCnt1Selected',0,'RXCnt2Selected',0,'TXCnt2Selected',0,'BothDirSelected',0,'DiffListsSelected',0,'MsgIdFormat',0,'TriggerPort',struct('Selected',0,'TriggerType','rising'),'EnablePortSelected',0),'ExcludeList12',struct('Count',0,'MsgList',struct('MsgId',0,'MsgName','empty','FromDBC',0)),'ExcludeList21',struct('Count',0,'MsgList',struct('MsgId',0,'MsgName','empty','FromDBC',0)),'Version',1,'general',struct('isFromLib',1)),'GroupId',struct('Group',{{'RTICAN'}},'No',1,'Behavior',{{'NAMECHANGE'}},'BlockType',{{'SINK'}},'NameChangeFlag',0),'GroupId2',struct('Group',{{'RTICAN'}},'No',2,'Behavior',{{'NAMECHANGE'}},'BlockType',{{'SINK'}},'NameChangeFlag',0),'SFcnRTICANMessage',struct('MsgIdFormat','STD','SampleTime',-1,'RXCnt1Selected','no','TXCnt1Selected','no','RXCnt2Selected','no','TXCnt2Selected','no','BothDirSelected','no','DiffListsSelected','no','EnablePortSelected','no','TriggerPort',struct('Selected','no','TriggerType','rising'),'ExcludeList12',struct('Count',0,'MsgList',struct('MsgId',0,'MsgName','empty','FromDBC',0)),'ExcludeList21',struct('Count',0,'MsgList',struct('MsgId',0,'MsgName','empty','FromDBC',0)),'BoardTypeNo',int32([4302 4302]),'BoardNo',int32([1 1]),'ControllerNo',int32([1 2]),'SFcnPortType','Scalar'),'TLCFileName','rtican_gw_message')
      settings: AttributesFormatString=Group Id: RTICAN1\n  SourceProductName=dSPACE RTI CAN Blockset
  Ground : Ground
  NET_CFG_PT1 : rtican/RTICAN Receive (RX)   Reserved1=[]  Reserved2=[]  Reserved3=[]  Reserved4=[]  SfcnMessage=[]  Msg_Struct=[]  BoardTypeNo=[]  BoardNo=[]  ChannelNo=[]  Parameters=[]  DialogFcn=[]  UnitName=[]  Revision=[]  UnitValues=[]  DSProperties=struct('RTI',struct('Version',uint32(5),'BlockType',struct('isSLSource',uint8(1),'isSLSink',uint8(1),'isHWSource',uint8(0),'isHWSink',uint8(0),'isSetup',uint8(0),'isInline',uint8(1),'isNonInline',uint8(0),'isInterrupt',uint8(0),'isChannelwise',uint8(0)),'IOBoardType','RTICAN','UnitType','MESSAGE','Identifier','RX','DialogType','MSVC','BlockSet','RTICAN','SlaveProcessor','CAN'))  RTIBlockInterface=struct('OutputPortsWidth',int32([1 1 1 1 1 1 1 1 1 1 1 1 1 1 1 1 1 1 1 1 1 1 1 1 1 1 1 1 1 1 1 1 1 1 1 1 1]),'OutputPortsActive',ones(1,37),'OutputPortsName',{{'NET_CFG_STAT_PT','NetCfg_ACC','NetCfg_ADCM','NetCfg_AHLM','NetCfg_VSIM_C','NetCfg_ASCM','NetCfg_CBC_PT','NetCfg_DTCM','NetCfg_ECM','NetCfg_EPS','NetCfg_ESM','NetCfg_ESC','NetCfg_EPB','NetCfg_RF_HUB','NetCfg_IC','NetCfg_DASM','NetCfg_FDCM','NetCfg_EPPM','NetCfg_ORC','NetCfg_PTS','NetCfg_SCCM','NetCfg_ELSD','NetCfg_TCM','NetCfg_TPM','NetCfg_PASS_PT','NetCfg_AFLS','NetCfg_ITBM','NetCfg_OCM','NetCfg_HaLF','NetCfg_BSMO','NetCfg_ESL','NetCfg_HCP','NetCfg_ANC','NetCfg_RHSC2',['RX status'],['RX time'],['RX delta time']}},'OutputPortsDataType',{{'SS_UINT8','SS_BOOLEAN','SS_BOOLEAN','SS_BOOLEAN','SS_BOOLEAN','SS_BOOLEAN','SS_BOOLEAN','SS_BOOLEAN','SS_BOOLEAN','SS_BOOLEAN','SS_BOOLEAN','SS_BOOLEAN','SS_BOOLEAN','SS_BOOLEAN','SS_BOOLEAN','SS_BOOLEAN','SS_BOOLEAN','SS_BOOLEAN','SS_BOOLEAN','SS_BOOLEAN','SS_BOOLEAN','SS_BOOLEAN','SS_BOOLEAN','SS_BOOLEAN','SS_BOOLEAN','SS_BOOLEAN','SS_BOOLEAN','SS_BOOLEAN','SS_BOOLEAN','SS_BOOLEAN','SS_BOOLEAN','SS_BOOLEAN','SS_BOOLEAN','SS_BOOLEAN','SS_DOUBLE','SS_DOUBLE','SS_DOUBLE'}},'OutputPortsLabel',{{'NET_CFG_STAT_PT','NetCfg_ACC','NetCfg_ADCM','NetCfg_AHLM','NetCfg_VSIM_C','NetCfg_ASCM','NetCfg_CBC_PT','NetCfg_DTCM','NetCfg_ECM','NetCfg_EPS','NetCfg_ESM','NetCfg_ESC','NetCfg_EPB','NetCfg_RF_HUB','NetCfg_IC','NetCfg_DASM','NetCfg_FDCM','NetCfg_EPPM','NetCfg_ORC','NetCfg_PTS','NetCfg_SCCM','NetCfg_ELSD','NetCfg_TCM','NetCfg_TPM','NetCfg_PASS_PT','NetCfg_AFLS','NetCfg_ITBM','NetCfg_OCM','NetCfg_HaLF','NetCfg_BSMO','NetCfg_ESL','NetCfg_HCP','NetCfg_ANC','NetCfg_RHSC2','','',''}},'OutputPortsLabelMode','ON','InputPortsWidth',int32(0),'InputPortsActive',0,'DialogFcn','rtican_message_interface_gui','BlockDisplay',{{'','center'}},'IconTransparency','on','ParameterTunableNames',{{}},'InitLevel',3,'BlockName',struct('Token',{{'NET_CFG_PT'}}),'SampleTime',{{-1}},'TriggerPort',{{'none'}},'EnablePort',{{'none'}})  RTIBlockParameters=struct('BoardTypeNo',{{1,'OFF',[]}},'BoardNo',{{1,'ON',[1 16]}},'ChannelNo',{{1,'ON',[1 2]}},'Parameters',{{struct('DataFileSupport',struct('DataFileSelectedMaster',1,'DataFileSelectedLocal',1,'DataFileName',['c:\intrepidcs\pacifica dbc\e4a_r4_ccan_cr11690_mod.dbc|'],'DataFileDate',{{{['26-Feb-2019 09:25:05']}}},'SelectedFile',['..\..\..\..\..\..\..\..\intrepidcs\pacifica dbc\e4a_r4_ccan_cr11690_mod.dbc']),'Options',struct('StatusSelected',1,'TimeSelected',1,'DeltaTimeSelected',1,'BytePortSelected',0,'MessageLengthSelected',0,'TriggerPort',struct('Selected',0,'TriggerType',0),'UserCoding',struct('Selected',0,'InterfaceFile','UserDecodingFile','FcnName','UserDecodeFcn','InportSelected',0,'InportWidth',1,'OutportSelected',0,'OutportWidth',1),'EnablePortSelected',0,'SignalOnPortnameSelected',1,'UseRXService',0),'Message',struct('MsgOnBlocknameSelected',1,'MsgName','NET_CFG_PT','MsgIdFormat',0,'MsgId',996,'MsgLength',8,'NumSignals',34,'SampleTime',-1,'Signal',struct('SgnName',{'NET_CFG_STAT_PT','NetCfg_ACC','NetCfg_ADCM','NetCfg_AHLM','NetCfg_VSIM_C','NetCfg_ASCM','NetCfg_CBC_PT','NetCfg_DTCM','NetCfg_ECM','NetCfg_EPS','NetCfg_ESM','NetCfg_ESC','NetCfg_EPB','NetCfg_RF_HUB','NetCfg_IC','NetCfg_DASM','NetCfg_FDCM','NetCfg_EPPM','NetCfg_ORC','NetCfg_PTS','NetCfg_SCCM','NetCfg_ELSD','NetCfg_TCM','NetCfg_TPM','NetCfg_PASS_PT','NetCfg_AFLS','NetCfg_ITBM','NetCfg_OCM','NetCfg_HaLF','NetCfg_BSMO','NetCfg_ESL','NetCfg_HCP','NetCfg_ANC','NetCfg_RHSC2'},'SgnStartBit',{0,2,3,4,5,6,7,8,9,10,11,12,13,14,15,16,17,18,19,20,23,24,25,26,27,28,29,30,31,36,37,38,39,44},'SgnLength',{2,1,1,1,1,1,1,1,1,1,1,1,1,1,1,1,1,1,1,1,1,1,1,1,1,1,1,1,1,1,1,1,1,1},'SgnType',{0,0,0,0,0,0,0,0,0,0,0,0,0,0,0,0,0,0,0,0,0,0,0,0,0,0,0,0,0,0,0,0,0,0},'ModeValue',{-1,-1,-1,-1,-1,-1,-1,-1,-1,-1,-1,-1,-1,-1,-1,-1,-1,-1,-1,-1,-1,-1,-1,-1,-1,-1,-1,-1,-1,-1,-1,-1,-1,-1},'DataType',{0,0,0,0,0,0,0,0,0,0,0,0,0,0,0,0,0,0,0,0,0,0,0,0,0,0,0,0,0,0,0,0,0,0},'ByteLayout',{0,0,0,0,0,0,0,0,0,0,0,0,0,0,0,0,0,0,0,0,0,0,0,0,0,0,0,0,0,0,0,0,0,0},'Factor',{1,1,1,1,1,1,1,1,1,1,1,1,1,1,1,1,1,1,1,1,1,1,1,1,1,1,1,1,1,1,1,1,1,1},'Offset',{0,0,0,0,0,0,0,0,0,0,0,0,0,0,0,0,0,0,0,0,0,0,0,0,0,0,0,0,0,0,0,0,0,0},'SgnComment',{{['Network configuration status']},{['Active Cruise Control (1=present)']},{['Active Damping Control Module (1=present)']},{['Automatic Headlamp Leveling Module (1=present)']},{['Vehicle System Interface Module (1=present)']},{['Air Suspension Control Module (1=present)']},{['Common Body Controller PT Bus (1=present)']},{['Drivetrain Control Module (1=present)']},{['Engine Control Module (1=present)']},{['Electric Power Steering (1=present)']},{['Electronic Shift Module (1=present)']},{['Electronic Stability Module / Anti-Lock Brake (1=present)']},{['Electric Park Brake Module (1=present)']},{['RF Hub Node (1=present)']},{['Instrument Cluster (1=present)']},{['Driver Assistance System Module (1=present)']},{['Final Drive Control Module (1=present)']},{['Elect. Pedestrian protection module (1=present)']},{['Occupant Restraint Controller (1=present)']},{['Parktronics System (1=present)']},{['Steering Column Control Module (1=present)']},{['Electric Limited Slip Differential (1=present)']},{['Automatic Transmission Controller (1=present)']},{['Tire Pressure Monitor (1=present)']},{['Personal Assistant Safety System Module PT Bus (1=present)']},{['Advanced Front Lighting System (1=present)']},{['Integrated Trailer Brake Module (1=present)']},{['Occupant Classification Module (1=present)']},{['Haptic Lane Feedback module (1=present)']},{['Brake System Module - OBD (1=present)']},{['Electric Steering Lock (1=present)']},{['Hybrid Control Processor (1=present)']},{['Active Noise Cancellation (1=present)']},{['RHSC2 module (1=present)']}},'SgnUnit',{'','','','','','','','','','','','','','','','','','','','','','','','','','','','','','','','','',''},'Min',{0,0,0,0,0,0,0,0,0,0,0,0,0,0,0,0,0,0,0,0,0,0,0,0,0,0,0,0,0,0,0,0,0,0},'Max',{0,0,0,0,0,0,0,0,0,0,0,0,0,0,0,0,0,0,0,0,0,0,0,0,0,0,0,0,0,0,0,0,0,0},'SLDataType',{'SS_UINT8','SS_BOOLEAN','SS_BOOLEAN','SS_BOOLEAN','SS_BOOLEAN','SS_BOOLEAN','SS_BOOLEAN','SS_BOOLEAN','SS_BOOLEAN','SS_BOOLEAN','SS_BOOLEAN','SS_BOOLEAN','SS_BOOLEAN','SS_BOOLEAN','SS_BOOLEAN','SS_BOOLEAN','SS_BOOLEAN','SS_BOOLEAN','SS_BOOLEAN','SS_BOOLEAN','SS_BOOLEAN','SS_BOOLEAN','SS_BOOLEAN','SS_BOOLEAN','SS_BOOLEAN','SS_BOOLEAN','SS_BOOLEAN','SS_BOOLEAN','SS_BOOLEAN','SS_BOOLEAN','SS_BOOLEAN','SS_BOOLEAN','SS_BOOLEAN','SS_BOOLEAN'}),'MsgIdNumFormat',0,'MsgComment',{{''}}),'Version',1.2,'general',struct('isFromLib',0)),'OFF',[]}},'GroupId',{{struct('Group',{{'RTICAN'}},'No',1,'Behavior',{{'NAMECHANGE'}},'BlockType',{{'SINK'}},'NameChangeFlag',0),'OFF',[]}},'SFcnRTICANMessage',{{struct('MsgType','RX','SFcnPortType','Scalar','MsgName','NET_CFG_PT','MsgIdFormat','STD','MsgId',996,'MsgLength',8,'NumSignals',34,'SampleTime',-1,'Signal',struct('SgnName',{'NET_CFG_STAT_PT','NetCfg_ACC','NetCfg_ADCM','NetCfg_AHLM','NetCfg_VSIM_C','NetCfg_ASCM','NetCfg_CBC_PT','NetCfg_DTCM','NetCfg_ECM','NetCfg_EPS','NetCfg_ESM','NetCfg_ESC','NetCfg_EPB','NetCfg_RF_HUB','NetCfg_IC','NetCfg_DASM','NetCfg_FDCM','NetCfg_EPPM','NetCfg_ORC','NetCfg_PTS','NetCfg_SCCM','NetCfg_ELSD','NetCfg_TCM','NetCfg_TPM','NetCfg_PASS_PT','NetCfg_AFLS','NetCfg_ITBM','NetCfg_OCM','NetCfg_HaLF','NetCfg_BSMO','NetCfg_ESL','NetCfg_HCP','NetCfg_ANC','NetCfg_RHSC2'},'SgnStartBit',{0,2,3,4,5,6,7,8,9,10,11,12,13,14,15,16,17,18,19,20,23,24,25,26,27,28,29,30,31,36,37,38,39,44},'SgnLength',{2,1,1,1,1,1,1,1,1,1,1,1,1,1,1,1,1,1,1,1,1,1,1,1,1,1,1,1,1,1,1,1,1,1},'SgnType',{'standard','standard','standard','standard','standard','standard','standard','standard','standard','standard','standard','standard','standard','standard','standard','standard','standard','standard','standard','standard','standard','standard','standard','standard','standard','standard','standard','standard','standard','standard','standard','standard','standard','standard'},'ModeValue',{-1,-1,-1,-1,-1,-1,-1,-1,-1,-1,-1,-1,-1,-1,-1,-1,-1,-1,-1,-1,-1,-1,-1,-1,-1,-1,-1,-1,-1,-1,-1,-1,-1,-1},'DataType',{['unsigned int'],['unsigned int'],['unsigned int'],['unsigned int'],['unsigned int'],['unsigned int'],['unsigned int'],['unsigned int'],['unsigned int'],['unsigned int'],['unsigned int'],['unsigned int'],['unsigned int'],['unsigned int'],['unsigned int'],['unsigned int'],['unsigned int'],['unsigned int'],['unsigned int'],['unsigned int'],['unsigned int'],['unsigned int'],['unsigned int'],['unsigned int'],['unsigned int'],['unsigned int'],['unsigned int'],['unsigned int'],['unsigned int'],['unsigned int'],['unsigned int'],['unsigned int'],['unsigned int'],['unsigned int']},'ByteLayout',{['little endian'],['little endian'],['little endian'],['little endian'],['little endian'],['little endian'],['little endian'],['little endian'],['little endian'],['little endian'],['little endian'],['little endian'],['little endian'],['little endian'],['little endian'],['little endian'],['little endian'],['little endian'],['little endian'],['little endian'],['little endian'],['little endian'],['little endian'],['little endian'],['little endian'],['little endian'],['little endian'],['little endian'],['little endian'],['little endian'],['little endian'],['little endian'],['little endian'],['little endian']},'Factor',{1,1,1,1,1,1,1,1,1,1,1,1,1,1,1,1,1,1,1,1,1,1,1,1,1,1,1,1,1,1,1,1,1,1},'Offset',{0,0,0,0,0,0,0,0,0,0,0,0,0,0,0,0,0,0,0,0,0,0,0,0,0,0,0,0,0,0,0,0,0,0},'SLDataType',{'SS_UINT8','SS_BOOLEAN','SS_BOOLEAN','SS_BOOLEAN','SS_BOOLEAN','SS_BOOLEAN','SS_BOOLEAN','SS_BOOLEAN','SS_BOOLEAN','SS_BOOLEAN','SS_BOOLEAN','SS_BOOLEAN','SS_BOOLEAN','SS_BOOLEAN','SS_BOOLEAN','SS_BOOLEAN','SS_BOOLEAN','SS_BOOLEAN','SS_BOOLEAN','SS_BOOLEAN','SS_BOOLEAN','SS_BOOLEAN','SS_BOOLEAN','SS_BOOLEAN','SS_BOOLEAN','SS_BOOLEAN','SS_BOOLEAN','SS_BOOLEAN','SS_BOOLEAN','SS_BOOLEAN','SS_BOOLEAN','SS_BOOLEAN','SS_BOOLEAN','SS_BOOLEAN'}),'StatusSelected','yes','TimeSelected','yes','DeltaTimeSelected','yes','BytePortSelected','no','MessageLengthSelected','no','TriggerPort',struct('Selected','no','TriggerType',0),'UserCoding',struct('Selected','no','InterfaceFile','UserDecodingFile','FcnName','UserDecodeFcn','InportSelected','no','InportWidth',1,'OutportSelected','no','OutportWidth',1),'EnablePortSelected','no','UseRXService','no','BoardType','DS1','BoardNo',1,'ControllerNo',1),'OFF',[]}},'TLCFileName',{{'rtican_rx_message','OFF',[]}})  RTISFcnParameters=struct('SFcnRTICANMessage','struct','TLCFileName','char')  RTIBlockParaDefault=struct('BoardTypeNo',4302,'BoardNo',1,'ChannelNo',1,'Parameters',struct('DataFileSupport',struct('DataFileSelectedMaster',0,'DataFileSelectedLocal',0,'DataFileName','','DataFileDate','','SelectedFile',['<no file selected>']),'Options',struct('StatusSelected',1,'TimeSelected',1,'DeltaTimeSelected',1,'BytePortSelected',0,'MessageLengthSelected',0,'TriggerPort',struct('Selected',0,'TriggerType','rising'),'UserCoding',struct('Selected',0,'InterfaceFile','UserDecodingFile','FcnName','UserDecodeFcn','InportSelected',0,'InportWidth',1,'OutportSelected',0,'OutportWidth',1),'EnablePortSelected',0,'SignalOnPortnameSelected',1,'UseRXService',0),'Message',struct('MsgOnBlocknameSelected',0,'MsgName',['RX Message'],'MsgIdFormat',0,'MsgId',100,'MsgLength',8,'NumSignals',1,'SampleTime',-1,'Signal',struct('SgnName',['RX signal'],'SgnStartBit',0,'SgnLength',8,'SgnType',0,'ModeValue',-1,'DataType',0,'SLDataType','SS_DOUBLE','ByteLayout',0,'Factor',1,'Offset',0,'Min',0,'Max',255,'SgnComment',{{}},'SgnUnit',''),'MsgIdNumFormat',0,'MsgComment',{{''}}),'Version',1.2,'general',struct('isFromLib',1)),'GroupId',struct('Group',{{'RTICAN'}},'No',1,'Behavior',{{'NAMECHANGE'}},'BlockType',{{'SINK'}},'NameChangeFlag',0),'SFcnRTICANMessage',struct('MsgType','RX','MsgName',['RX Message'],'MsgIdFormat','STD','MsgId',100,'MsgLength',8,'NumSignals',1,'SampleTime',-1,'Signal',struct('SgnName',['RX signal'],'SgnStartBit',0,'SgnLength',8,'SgnType','standard','ModeValue',-1,'DataType',['unsigned int'],'ByteLayout',['little endian'],'SLDataType','SS_DOUBLE','Factor',1,'Offset',0),'StatusSelected','yes','TimeSelected','yes','DeltaTimeSelected','yes','BytePortSelected','no','MessageLengthSelected','no','EnablePortSelected','no','UserCoding',struct('Selected','no','InterfaceFile','UserDecodingFile','FcnName','UserDecodeFcn','InportSelected','no','InportWidth',1,'OutportSelected','no','OutportWidth',1),'TriggerPort',struct('Selected','no','TriggerType','rising'),'UseRXService','no','BoardType','DS4302','BoardNo',1,'ControllerNo',1,'SFcnPortType','Scalar'),'TLCFileName','rtican_rx_message')
      settings: AttributesFormatString=Group Id: RTICAN1\n  SourceProductName=dSPACE RTI CAN Blockset
  NET_CFG_PT2 : rtican/RTICAN Transmit (TX)   Reserved1=[]  Reserved2=[]  Reserved3=[]  Reserved4=[]  SfcnMessage=[]  Msg_Struct=[]  BoardTypeNo=[]  BoardNo=[]  ChannelNo=[]  Parameters=[]  DialogFcn=[]  UnitName=[]  Revision=[]  UnitValues=[]  DSProperties=struct('RTI',struct('Version',uint32(5),'BlockType',struct('isSLSource',uint8(1),'isSLSink',uint8(1),'isHWSource',uint8(0),'isHWSink',uint8(0),'isSetup',uint8(0),'isInline',uint8(1),'isNonInline',uint8(0),'isInterrupt',uint8(0),'isChannelwise',uint8(0)),'IOBoardType','RTICAN','UnitType','MESSAGE','Identifier','TX','DialogType','MSVC','BlockSet','RTICAN','SlaveProcessor','CAN'))  RTIBlockInterface=struct('InputPortsWidth',int32([1 1 1 1 1 1 1 1 1 1 1 1 1 1 1 1 1 1 1 1 1 1 1 1 1 1 1 1 1 1 1 1 1 1]),'InputPortsActive',ones(1,34),'InputPortsName',{{'NET_CFG_STAT_PT','NetCfg_ACC','NetCfg_ADCM','NetCfg_AHLM','NetCfg_VSIM_C','NetCfg_ASCM','NetCfg_CBC_PT','NetCfg_DTCM','NetCfg_ECM','NetCfg_EPS','NetCfg_ESM','NetCfg_ESC','NetCfg_EPB','NetCfg_RF_HUB','NetCfg_IC','NetCfg_DASM','NetCfg_FDCM','NetCfg_EPPM','NetCfg_ORC','NetCfg_PTS','NetCfg_SCCM','NetCfg_ELSD','NetCfg_TCM','NetCfg_TPM','NetCfg_PASS_PT','NetCfg_AFLS','NetCfg_ITBM','NetCfg_OCM','NetCfg_HaLF','NetCfg_BSMO','NetCfg_ESL','NetCfg_HCP','NetCfg_ANC','NetCfg_RHSC2'}},'InputPortsDataType',{{'SS_UINT8','SS_BOOLEAN','SS_BOOLEAN','SS_BOOLEAN','SS_BOOLEAN','SS_BOOLEAN','SS_BOOLEAN','SS_BOOLEAN','SS_BOOLEAN','SS_BOOLEAN','SS_BOOLEAN','SS_BOOLEAN','SS_BOOLEAN','SS_BOOLEAN','SS_BOOLEAN','SS_BOOLEAN','SS_BOOLEAN','SS_BOOLEAN','SS_BOOLEAN','SS_BOOLEAN','SS_BOOLEAN','SS_BOOLEAN','SS_BOOLEAN','SS_BOOLEAN','SS_BOOLEAN','SS_BOOLEAN','SS_BOOLEAN','SS_BOOLEAN','SS_BOOLEAN','SS_BOOLEAN','SS_BOOLEAN','SS_BOOLEAN','SS_BOOLEAN','SS_BOOLEAN'}},'OutputPortsWidth',int32([1 1 1 1]),'OutputPortsActive',[1 1 1 1],'OutputPortsName',{{['TX status'],['TX time'],['TX delta time'],['TX delay time']}},'DialogFcn','rtican_message_interface_gui','BlockDisplay',{{'','center'}},'IconTransparency','on','InitLevel',3,'BlockName',struct('Token',{{'NET_CFG_PT'}}),'SampleTime',{{-1}},'TriggerPort',{{'none'}},'EnablePort',{{'yes'}})  RTIBlockParameters=struct('BoardTypeNo',{{1,'OFF',[]}},'BoardNo',{{1,'ON',[1 16]}},'ChannelNo',{{1,'ON',[1 2]}},'Parameters',{{struct('DataFileSupport',struct('DataFileSelectedMaster',1,'DataFileSelectedLocal',1,'DataFileName',['c:\intrepidcs\pacifica dbc\e4a_r4_ccan_cr11690_mod.dbc|'],'DataFileDate',{{{['26-Feb-2019 09:25:05']}}},'SelectedFile',['..\..\..\..\..\..\..\..\intrepidcs\pacifica dbc\e4a_r4_ccan_cr11690_mod.dbc']),'Options',struct('StatusSelected',1,'TimeSelected',1,'DeltaTimeSelected',1,'DelayTimeSelected',1,'DelayTimeTXCommandSelected',0,'EncodeSetUnusedBitsToOne',0,'EnableMsgLoopback',0,'TriggerPort',struct('Selected',0,'TriggerType',0),'EnablePortSelected',1,'SignalOnPortnameSelected',1,'UserCoding',struct('Selected',1,'InterfaceFile','UserEncodingFile','FcnName','Message_CRC_Encoder','InportSelected',0,'InportWidth',1,'OutportSelected',0,'OutportWidth',1),'TerminationMsg',struct('Selected',0,'Byte0_7','0'),'InitialMsg',struct('Selected',0,'Byte0_7','0')),'Message',struct('MsgOnBlocknameSelected',1,'MsgName','NET_CFG_PT','MsgIdFormat',0,'MsgId',996,'MsgLength',8,'NumSignals',34,'SampleTime',-1,'StartTime',struct('Selected',0,'Value',7),'AutoRepeatTime',struct('Selected',0,'Value',0.1),'Timeout',struct('Selected',0,'Value',0.1),'DelayTime',struct('Selected',0,'Value',0.1),'Signal',struct('SgnName',{'NET_CFG_STAT_PT','NetCfg_ACC','NetCfg_ADCM','NetCfg_AHLM','NetCfg_VSIM_C','NetCfg_ASCM','NetCfg_CBC_PT','NetCfg_DTCM','NetCfg_ECM','NetCfg_EPS','NetCfg_ESM','NetCfg_ESC','NetCfg_EPB','NetCfg_RF_HUB','NetCfg_IC','NetCfg_DASM','NetCfg_FDCM','NetCfg_EPPM','NetCfg_ORC','NetCfg_PTS','NetCfg_SCCM','NetCfg_ELSD','NetCfg_TCM','NetCfg_TPM','NetCfg_PASS_PT','NetCfg_AFLS','NetCfg_ITBM','NetCfg_OCM','NetCfg_HaLF','NetCfg_BSMO','NetCfg_ESL','NetCfg_HCP','NetCfg_ANC','NetCfg_RHSC2'},'SgnStartBit',{0,2,3,4,5,6,7,8,9,10,11,12,13,14,15,16,17,18,19,20,23,24,25,26,27,28,29,30,31,36,37,38,39,44},'SgnLength',{2,1,1,1,1,1,1,1,1,1,1,1,1,1,1,1,1,1,1,1,1,1,1,1,1,1,1,1,1,1,1,1,1,1},'SgnType',{0,0,0,0,0,0,0,0,0,0,0,0,0,0,0,0,0,0,0,0,0,0,0,0,0,0,0,0,0,0,0,0,0,0},'ModeValue',{-1,-1,-1,-1,-1,-1,-1,-1,-1,-1,-1,-1,-1,-1,-1,-1,-1,-1,-1,-1,-1,-1,-1,-1,-1,-1,-1,-1,-1,-1,-1,-1,-1,-1},'DataType',{0,0,0,0,0,0,0,0,0,0,0,0,0,0,0,0,0,0,0,0,0,0,0,0,0,0,0,0,0,0,0,0,0,0},'ByteLayout',{0,0,0,0,0,0,0,0,0,0,0,0,0,0,0,0,0,0,0,0,0,0,0,0,0,0,0,0,0,0,0,0,0,0},'Factor',{1,1,1,1,1,1,1,1,1,1,1,1,1,1,1,1,1,1,1,1,1,1,1,1,1,1,1,1,1,1,1,1,1,1},'Offset',{0,0,0,0,0,0,0,0,0,0,0,0,0,0,0,0,0,0,0,0,0,0,0,0,0,0,0,0,0,0,0,0,0,0},'SgnComment',{{['Network configuration status']},{['Active Cruise Control (1=present)']},{['Active Damping Control Module (1=present)']},{['Automatic Headlamp Leveling Module (1=present)']},{['Vehicle System Interface Module (1=present)']},{['Air Suspension Control Module (1=present)']},{['Common Body Controller PT Bus (1=present)']},{['Drivetrain Control Module (1=present)']},{['Engine Control Module (1=present)']},{['Electric Power Steering (1=present)']},{['Electronic Shift Module (1=present)']},{['Electronic Stability Module / Anti-Lock Brake (1=present)']},{['Electric Park Brake Module (1=present)']},{['RF Hub Node (1=present)']},{['Instrument Cluster (1=present)']},{['Driver Assistance System Module (1=present)']},{['Final Drive Control Module (1=present)']},{['Elect. Pedestrian protection module (1=present)']},{['Occupant Restraint Controller (1=present)']},{['Parktronics System (1=present)']},{['Steering Column Control Module (1=present)']},{['Electric Limited Slip Differential (1=present)']},{['Automatic Transmission Controller (1=present)']},{['Tire Pressure Monitor (1=present)']},{['Personal Assistant Safety System Module PT Bus (1=present)']},{['Advanced Front Lighting System (1=present)']},{['Integrated Trailer Brake Module (1=present)']},{['Occupant Classification Module (1=present)']},{['Haptic Lane Feedback module (1=present)']},{['Brake System Module - OBD (1=present)']},{['Electric Steering Lock (1=present)']},{['Hybrid Control Processor (1=present)']},{['Active Noise Cancellation (1=present)']},{['RHSC2 module (1=present)']}},'SgnUnit',{'','','','','','','','','','','','','','','','','','','','','','','','','','','','','','','','','',''},'Min',{0,0,0,0,0,0,0,0,0,0,0,0,0,0,0,0,0,0,0,0,0,0,0,0,0,0,0,0,0,0,0,0,0,0},'Max',{0,0,0,0,0,0,0,0,0,0,0,0,0,0,0,0,0,0,0,0,0,0,0,0,0,0,0,0,0,0,0,0,0,0},'SLDataType',{'SS_UINT8','SS_BOOLEAN','SS_BOOLEAN','SS_BOOLEAN','SS_BOOLEAN','SS_BOOLEAN','SS_BOOLEAN','SS_BOOLEAN','SS_BOOLEAN','SS_BOOLEAN','SS_BOOLEAN','SS_BOOLEAN','SS_BOOLEAN','SS_BOOLEAN','SS_BOOLEAN','SS_BOOLEAN','SS_BOOLEAN','SS_BOOLEAN','SS_BOOLEAN','SS_BOOLEAN','SS_BOOLEAN','SS_BOOLEAN','SS_BOOLEAN','SS_BOOLEAN','SS_BOOLEAN','SS_BOOLEAN','SS_BOOLEAN','SS_BOOLEAN','SS_BOOLEAN','SS_BOOLEAN','SS_BOOLEAN','SS_BOOLEAN','SS_BOOLEAN','SS_BOOLEAN'}),'MsgIdNumFormat',0,'MsgComment',{{''}}),'Version',1.2,'general',struct('isFromLib',0)),'OFF',[]}},'GroupId',{{struct('Group',{{'RTICAN'}},'No',1,'Behavior',{{'NAMECHANGE'}},'BlockType',{{'SINK'}},'NameChangeFlag',0),'OFF',[]}},'SFcnRTICANMessage',{{struct('MsgType','TX','SFcnPortType','Scalar','MsgName','NET_CFG_PT','MsgIdFormat','STD','MsgId',996,'MsgLength',8,'NumSignals',34,'SampleTime',-1,'StartTime',struct('Selected','no','Value',7),'AutoRepeatTime',struct('Selected','no','Value',0.1),'Timeout',struct('Selected','no','Value',0.1),'Signal',struct('SgnName',{'NET_CFG_STAT_PT','NetCfg_ACC','NetCfg_ADCM','NetCfg_AHLM','NetCfg_VSIM_C','NetCfg_ASCM','NetCfg_CBC_PT','NetCfg_DTCM','NetCfg_ECM','NetCfg_EPS','NetCfg_ESM','NetCfg_ESC','NetCfg_EPB','NetCfg_RF_HUB','NetCfg_IC','NetCfg_DASM','NetCfg_FDCM','NetCfg_EPPM','NetCfg_ORC','NetCfg_PTS','NetCfg_SCCM','NetCfg_ELSD','NetCfg_TCM','NetCfg_TPM','NetCfg_PASS_PT','NetCfg_AFLS','NetCfg_ITBM','NetCfg_OCM','NetCfg_HaLF','NetCfg_BSMO','NetCfg_ESL','NetCfg_HCP','NetCfg_ANC','NetCfg_RHSC2'},'SgnStartBit',{0,2,3,4,5,6,7,8,9,10,11,12,13,14,15,16,17,18,19,20,23,24,25,26,27,28,29,30,31,36,37,38,39,44},'SgnLength',{2,1,1,1,1,1,1,1,1,1,1,1,1,1,1,1,1,1,1,1,1,1,1,1,1,1,1,1,1,1,1,1,1,1},'SgnType',{'standard','standard','standard','standard','standard','standard','standard','standard','standard','standard','standard','standard','standard','standard','standard','standard','standard','standard','standard','standard','standard','standard','standard','standard','standard','standard','standard','standard','standard','standard','standard','standard','standard','standard'},'ModeValue',{-1,-1,-1,-1,-1,-1,-1,-1,-1,-1,-1,-1,-1,-1,-1,-1,-1,-1,-1,-1,-1,-1,-1,-1,-1,-1,-1,-1,-1,-1,-1,-1,-1,-1},'DataType',{['unsigned int'],['unsigned int'],['unsigned int'],['unsigned int'],['unsigned int'],['unsigned int'],['unsigned int'],['unsigned int'],['unsigned int'],['unsigned int'],['unsigned int'],['unsigned int'],['unsigned int'],['unsigned int'],['unsigned int'],['unsigned int'],['unsigned int'],['unsigned int'],['unsigned int'],['unsigned int'],['unsigned int'],['unsigned int'],['unsigned int'],['unsigned int'],['unsigned int'],['unsigned int'],['unsigned int'],['unsigned int'],['unsigned int'],['unsigned int'],['unsigned int'],['unsigned int'],['unsigned int'],['unsigned int']},'ByteLayout',{['little endian'],['little endian'],['little endian'],['little endian'],['little endian'],['little endian'],['little endian'],['little endian'],['little endian'],['little endian'],['little endian'],['little endian'],['little endian'],['little endian'],['little endian'],['little endian'],['little endian'],['little endian'],['little endian'],['little endian'],['little endian'],['little endian'],['little endian'],['little endian'],['little endian'],['little endian'],['little endian'],['little endian'],['little endian'],['little endian'],['little endian'],['little endian'],['little endian'],['little endian']},'Factor',{1,1,1,1,1,1,1,1,1,1,1,1,1,1,1,1,1,1,1,1,1,1,1,1,1,1,1,1,1,1,1,1,1,1},'Offset',{0,0,0,0,0,0,0,0,0,0,0,0,0,0,0,0,0,0,0,0,0,0,0,0,0,0,0,0,0,0,0,0,0,0},'SLDataType',{'SS_UINT8','SS_BOOLEAN','SS_BOOLEAN','SS_BOOLEAN','SS_BOOLEAN','SS_BOOLEAN','SS_BOOLEAN','SS_BOOLEAN','SS_BOOLEAN','SS_BOOLEAN','SS_BOOLEAN','SS_BOOLEAN','SS_BOOLEAN','SS_BOOLEAN','SS_BOOLEAN','SS_BOOLEAN','SS_BOOLEAN','SS_BOOLEAN','SS_BOOLEAN','SS_BOOLEAN','SS_BOOLEAN','SS_BOOLEAN','SS_BOOLEAN','SS_BOOLEAN','SS_BOOLEAN','SS_BOOLEAN','SS_BOOLEAN','SS_BOOLEAN','SS_BOOLEAN','SS_BOOLEAN','SS_BOOLEAN','SS_BOOLEAN','SS_BOOLEAN','SS_BOOLEAN'}),'StatusSelected','yes','TimeSelected','yes','DeltaTimeSelected','yes','DelayTimeSelected','yes','DelayTimeTXCommandSelected','no','EncodeSetUnusedBitsToOne','no','EnableMsgLoopback','no','TriggerPort',struct('Selected','no','TriggerType',0),'EnablePortSelected','yes','UserCoding',struct('Selected','yes','InterfaceFile','UserEncodingFile','FcnName','Message_CRC_Encoder','InportSelected','no','InportWidth',1,'OutportSelected','no','OutportWidth',1),'TerminationMsg',struct('Selected','no','Byte0','0x00','Byte1','0x00','Byte2','0x00','Byte3','0x00','Byte4','0x00','Byte5','0x00','Byte6','0x00','Byte7','0x00'),'InitialMsg',struct('Selected','no','Byte0','0x00','Byte1','0x00','Byte2','0x00','Byte3','0x00','Byte4','0x00','Byte5','0x00','Byte6','0x00','Byte7','0x00'),'BoardType','DS1','BoardNo',1,'ControllerNo',1),'OFF',[]}},'TLCFileName',{{'rtican_tx_message','OFF',[]}})  RTISFcnParameters=struct('SFcnRTICANMessage','struct','TLCFileName','char')  RTIBlockParaDefault=struct('BoardTypeNo',4302,'BoardNo',1,'ChannelNo',1,'Parameters',struct('DataFileSupport',struct('DataFileSelectedMaster',0,'DataFileSelectedLocal',0,'DataFileName','','DataFileDate','','SelectedFile',['<no file selected>']),'Options',struct('StatusSelected',1,'TimeSelected',1,'DeltaTimeSelected',1,'DelayTimeSelected',1,'DelayTimeTXCommandSelected',0,'EncodeSetUnusedBitsToOne',0,'EnableMsgLoopback',0,'TriggerPort',struct('Selected',0,'TriggerType','rising'),'EnablePortSelected',0,'SignalOnPortnameSelected',1,'UserCoding',struct('Selected',0,'InterfaceFile','UserEncodingFile','FcnName','UserEncodeFcn','InportSelected',0,'InportWidth',1,'OutportSelected',0,'OutportWidth',1),'TerminationMsg',struct('Selected',0,'Byte0_7','0'),'InitialMsg',struct('Selected',0,'Byte0_7','0')),'Message',struct('MsgOnBlocknameSelected',0,'MsgName',['TX Message'],'MsgIdFormat',0,'MsgId',100,'MsgLength',8,'NumSignals',1,'SampleTime',-1,'StartTime',struct('Selected',0,'Value',0),'AutoRepeatTime',struct('Selected',0,'Value',0.1),'Timeout',struct('Selected',0,'Value',0.1),'DelayTime',struct('Selected',0,'Value',0.1),'Signal',struct('SgnName',['TX signal'],'SgnStartBit',0,'SgnLength',8,'SgnType',0,'ModeValue',-1,'DataType',0,'SLDataType','SS_DOUBLE','ByteLayout',0,'Factor',1,'Offset',0,'Min',0,'Max',255,'SgnComment',{{}},'SgnUnit',''),'MsgIdNumFormat',0,'MsgComment',{{''}}),'Version',1.2,'general',struct('isFromLib',1)),'GroupId',struct('Group',{{'RTICAN'}},'No',1,'Behavior',{{'NAMECHANGE'}},'BlockType',{{'SINK'}},'NameChangeFlag',0),'SFcnRTICANMessage',struct('MsgType','TX','MsgName',['TX Message'],'MsgIdFormat','STD','MsgId',100,'MsgLength',2,'NumSignals',1,'SampleTime',-1,'StartTime',struct('Selected','no','Value',0),'AutoRepeatTime',struct('Selected','no','Value',0.1),'Timeout',struct('Selected','no','Value',0.1),'DelayTime',struct('Selected','no','Value',0.1),'Signal',struct('SgnName',['TX signal'],'SgnStartBit',0,'SgnLength',8,'SgnType','standard','ModeValue',-1,'DataType',['unsigned int'],'ByteLayout',['little endian'],'SLDataType','SS_DOUBLE','Factor',1,'Offset',0),'StatusSelected','yes','TimeSelected','yes','DeltaTimeSelected','yes','DelayTimeSelected','yes','EnablePortSelected','no','EnableMsgLoopback','no','DelayTimeTXCommandSelected','no','EncodeSetUnusedBitsToOne','no','UserCoding',struct('Selected','no','InterfaceFile','UserDecodingFile','FcnName','UserDecodeFcn','InportSelected','no','InportWidth',1,'OutportSelected','no','OutportWidth',1),'TerminationMsg',struct('Selected','no','Byte0','0x00','Byte1','0x00','Byte2','0x00','Byte3','0x00','Byte4','0x00','Byte5','0x00','Byte6','0x00','Byte7','0x00'),'InitialMsg',struct('Selected','no','Byte0','0x00','Byte1','0x00','Byte2','0x00','Byte3','0x00','Byte4','0x00','Byte5','0x00','Byte6','0x00','Byte7','0x00'),'TriggerPort',struct('Selected','no','TriggerType','rising'),'BoardType','DS4302','BoardNo',1,'ControllerNo',1,'SFcnPortType','Scalar'),'TLCFileName','rtican_tx_message')
      settings: AttributesFormatString=Group Id: RTICAN1\n  SourceProductName=dSPACE RTI CAN Blockset
  RTI Data : Subsystem  Tag=struct('RTIDataServer',struct('RTIDataServerVs','2','RTIModelDescription','struct(''main'',''AEB_Gateway_Only'',''sub'','''',''isMp'',0)'))  LoadFcn="if exist('rtidc'), try,  rtidc('DataHostBlockClbLoad', gcbh); catch, disp(['Warning: ''LoadFcn'' for RTI Data block failed: ' lasterr]); end, end,"  mask(RTI_DATA_HOST){}
      mask help:
      | RTI Data Block.
      | This block is used by RTI to store internal model-dependent data.
      | Please keep this block on the root level of the model. Deleting this block will result in data loss.
      |
      | NEVER DELETE OR COPY THIS BLOCK!
      settings: CopyFcn="if exist('rtidc'), try,  rtidc('DataHostBlockClbCopy', gcbh); catch, disp(['Warning: ''CopyFcn'' for RTI Data block failed: ' lasterr]); end, end,"  DeleteFcn="if exist('rtidc'), try,  rtidc('DataHostBlockClbDelete', gcbh); catch, disp(['Warning: ''DeleteFcn'' for RTI Data block failed: ' lasterr]); end, end,"  ModelCloseFcn="if exist('rtidc'), try,  rtidc('DataHostBlockClbModelClose', gcbh); catch, disp(['Warning: ''ModelCloseFcn'' for RTI Data block failed: ' lasterr]); end, end,"  PreSaveFcn="if exist('rtidc'), try,  rtidc('DataHostBlockClbPreSave', gcbh); catch, disp(['Warning: ''PreSaveFcn'' for RTI Data block failed: ' lasterr]); end, end,"  PostSaveFcn="if exist('rtidc'), try,  rtidc('DataHostBlockClbPostSave', gcbh); catch, disp(['Warning: ''PostSaveFcn'' for RTI Data block failed: ' lasterr]); end, end,"  NameChangeFcn="if exist('rtidc'), try,  rtidc('DataHostBlockClbNameChange', gcbh); catch, disp(['Warning: ''NameChangeFcn'' for RTI Data block failed: ' lasterr]); end, end,"
      mask Help:
      | RTI Data Block.
      | This block is used by RTI to store internal model-dependent data.
      | Please keep this block on the root level of the model. Deleting this block will result in data loss.
      | 
      | NEVER DELETE OR COPY THIS BLOCK!
      mask Display:
      | text(0.5, 0.5, 'RTI Data', 'HorizontalAlignment', 'center');
      | plot([1 0]);
  wires:
  Constant/1 -> ESP_A2/3
  Constant1/1 -> ESP_A2/6
  Constant2/1 -> ESP_A2/5
  Constant3/1 -> ESP_A2/4
  Constant4/1 -> ESP_A2/8
  Constant5/1 -> ESP_A2/1
  Ground/1 -> ESP_A2/10
  Constant7/1 -> ESP_A2/11
  ESP_A21/14 -> ESP_A2/Enable
  ESP_A21/12 -> Data Type Conversion/1  "MC_ENG_RQ_ESC"
  NET_CFG_PT1/1 -> NET_CFG_PT2/1  "NET_CFG_STAT_PT"
  NET_CFG_PT1/2 -> NET_CFG_PT2/2  "NetCfg_ACC"
  NET_CFG_PT1/3 -> NET_CFG_PT2/3  "NetCfg_ADCM"
  NET_CFG_PT1/4 -> NET_CFG_PT2/4  "NetCfg_AHLM"
  NET_CFG_PT1/5 -> NET_CFG_PT2/5  "NetCfg_VSIM_C"
  NET_CFG_PT1/6 -> NET_CFG_PT2/6  "NetCfg_ASCM"
  NET_CFG_PT1/7 -> NET_CFG_PT2/7  "NetCfg_CBC_PT"
  NET_CFG_PT1/8 -> NET_CFG_PT2/8  "NetCfg_DTCM"
  NET_CFG_PT1/9 -> NET_CFG_PT2/9  "NetCfg_ECM"
  NET_CFG_PT1/10 -> NET_CFG_PT2/10  "NetCfg_EPS"
  NET_CFG_PT1/11 -> NET_CFG_PT2/11  "NetCfg_ESM"
  NET_CFG_PT1/12 -> NET_CFG_PT2/12  "NetCfg_ESC"
  NET_CFG_PT1/13 -> NET_CFG_PT2/13  "NetCfg_EPB"
  NET_CFG_PT1/14 -> NET_CFG_PT2/14  "NetCfg_RF_HUB"
  NET_CFG_PT1/15 -> NET_CFG_PT2/15  "NetCfg_IC"
  NET_CFG_PT1/16 -> NET_CFG_PT2/16  "NetCfg_DASM"
  NET_CFG_PT1/17 -> NET_CFG_PT2/17  "NetCfg_FDCM"
  NET_CFG_PT1/18 -> NET_CFG_PT2/18  "NetCfg_EPPM"
  NET_CFG_PT1/19 -> NET_CFG_PT2/19  "NetCfg_ORC"
  NET_CFG_PT1/20 -> NET_CFG_PT2/20  "NetCfg_PTS"
  NET_CFG_PT1/21 -> NET_CFG_PT2/21  "NetCfg_SCCM"
  NET_CFG_PT1/22 -> NET_CFG_PT2/22  "NetCfg_ELSD"
  NET_CFG_PT1/23 -> NET_CFG_PT2/23  "NetCfg_TCM"
  NET_CFG_PT1/24 -> NET_CFG_PT2/24  "NetCfg_TPM"
  NET_CFG_PT1/25 -> NET_CFG_PT2/25  "NetCfg_PASS_PT"
  NET_CFG_PT1/26 -> NET_CFG_PT2/26  "NetCfg_AFLS"
  NET_CFG_PT1/27 -> NET_CFG_PT2/27  "NetCfg_ITBM"
  NET_CFG_PT1/28 -> NET_CFG_PT2/28  "NetCfg_OCM"
  Constant6/1 -> NET_CFG_PT2/29  "NetCfg_HaLF"
  NET_CFG_PT1/30 -> NET_CFG_PT2/30  "NetCfg_BSMO"
  NET_CFG_PT1/31 -> NET_CFG_PT2/31  "NetCfg_ESL"
  NET_CFG_PT1/32 -> NET_CFG_PT2/32  "NetCfg_HCP"
  NET_CFG_PT1/33 -> NET_CFG_PT2/33  "NetCfg_ANC"
  NET_CFG_PT1/34 -> NET_CFG_PT2/34  "NetCfg_RHSC2"
  NET_CFG_PT1/35 -> NET_CFG_PT2/Enable
  Data Type Conversion/1 -> ESP_A2/12
